simulink model "ds_simple_twozone"  (R2020a)
settings: Solver=ode1be  StartTime=0.0  StopTime=Inf  FixedStep=0.001  RelTol=1e-3
PostLoadFcn:
  | if any(exist('dsrtsu_mdlpostloadfcn', 'file') ~= 0), dsrtsu_mdlpostloadfcn('Execute', bdroot); end
InitFcn:
  | , if any(exist('rtifpga_mdlclblib', 'file') ~= 0), rtifpga_mdlclblib('Init', bdroot); end,
  | , if any(exist('dsmpb_private', 'file') ~= 0), dsmpb_private('dsmpb_mdlclblib', 'Init', bdroot); end,
libraries: neural x7, dsmpblib x7
(part 2 of 3)

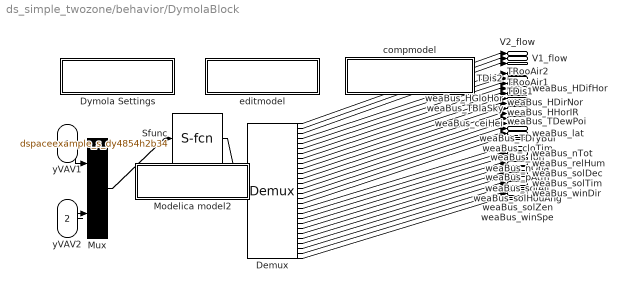
== system ds_simple_twozone/behavior/DymolaBlock ==
  yVAV1 : Inport
  yVAV2 : Inport  Port=2
  Demux : Demux  Outputs=[1;1;1;1;1;1;1;1;1;1;1;1;1;1;1;1;1;1;1;1;1;1;1;1;1;1;1;1]
  Dymola Settings : Subsystem  mask{ModelName=dSpaceExample.SimpleTwoZone, MoFileName=D:/github/dspace-modelica-example/dSpaceExample/SimpleTwoZone.mo, dSpace=, BusConnector=0, ResultFile=[], ResultFileOnline=[], ResultDt=[], Libs=:, bigobj=[], ImportFolder=[], guimode=[], ModelName2=[], forRuntime=[], MEXLoad=[], omitDescription=[], ResultName=dspaceexample_s_dy4854h2b34}
      mask prompts: ModelName "Name of Dymola model"; MoFileName "File Name (including .mo)"; ResultFile "Create Result"; ResultFileOnline "Load result"; ResultDt "Result min dt"; Libs "Used Libraries"; bigobj "Compiler flag /bigobj"; ImportFolder "Import folder"; guimode "GUI mode flag"; ModelName2 "Model name for import mode"; forRuntime "Runtime export"; MEXLoad "Compiled S-function"; omitDescription "Omit description strings"; ResultName "Name of result file"
      mask Display: disp('Dymola Settings');
  Modelica model2 : Subsystem
      mask Display: disp('Change parameters');
  Mux : Mux  Inputs=[1;1]
  Sfunc : S-Function  Tag=4854h2b34  FunctionName=dspaceexample_s_dy4854h2b34  Parameters=[VRoo;vav1_vav_sta_default_p;vav1_vav_sta_default_T;vav1_vav_sta_default_X;vav1_vav_riseTime;vav1_vav_y_start;vav1_vav_filter_gain;vav1_vav_filter_A_ripple;vav1_vav_filter_f_min;vav1_vav_filter_normalize10;vav1_vav_filter_x_start;vav1_vav_filter_u_nominal;vav1_vav_use_deltaM;vav1_vav_deltaM;vav1_vav_roundDuct;vav1_vav_ReC;vav1_vav_a;vav1_vav_b;vav1_vav_yL;vav1_vav_yU;vav1_vav_k1;vav1_vav_l;vav1_vav_l2;vav1_vav_deltax;vav1_vav_y_min;vav1_terHea_bal1_preDro_s26;vav1_terHea_bal1_preDro_s27;vav1_terHea_bal1_preDro_s28;vav1_terHea_bal2_preDro_s29;vav1_terHea_bal2_preDro_s30;vav1_terHea_delta;vav1_terHea_T_a1_nominal;vav1_terHea_T_a2_nominal;vav1_terHea_r_nominal;vav1_terHea_hA_n_w;vav1_terHea_hA_n_a;vav1_terHea_hA_T0_w;vav1_terHea_hA_T0_a;vav1_sinTer_X;vav1_sinTer_p;vav1_sinTer_T;vav1_souTer_X;vav1_souTer_m_flow;vav1_souTer_T;zer_k;zon1_S_;zon1_E_;zon1_W_;zon1_N_;zon1_matExtWal_absIR_a;zon1_matExtWal_absIR_b;zon1_matExtWal_absSol_a;zon1_matExtWal_absSol_b;zon1_matExtWal_roughness_54;zon1_matFlo_absIR_a;zon1_matFlo_absIR_b;zon1_matFlo_absSol_a;zon1_matFlo_absSol_b;zon1_matFlo_roughness_a;zon1_roof_absIR_a;zon1_roof_absIR_b;zon1_roof_absSol_a;zon1_roof_absSol_b;zon1_roof_roughness_a;zon1_window600_glass_1__x;zon1_window600_glass_1__k;zon1_window600_glass_1__t67;zon1_window600_glass_1__r68;zon1_window600_glass_1__r69;zon1_window600_glass_1__t70;zon1_window600_glass_1__a71;zon1_window600_glass_1__a72;zon1_window600_glass_2__x;zon1_window600_glass_2__k;zon1_window600_glass_2__t75;zon1_window600_glass_2__r76;zon1_window600_glass_2__r77;zon1_window600_glass_2__t78;zon1_window600_glass_2__a79;zon1_window600_glass_2__a80;zon1_window600_gas_1__x;zon1_window600_gas_1__a_k;zon1_window600_gas_1__b_k;zon1_window600_gas_1__a_m84;zon1_window600_gas_1__b_m85;zon1_window600_gas_1__a_c;zon1_window600_gas_1__b_c;zon1_window600_gas_1__MM;zon1_window600_gas_1__P0;zon1_window600_shade_tauS90;zon1_window600_shade_tauS91;zon1_window600_shade_rhoS92;zon1_window600_shade_rhoS93;zon1_window600_shade_absI94;zon1_window600_shade_absI95;zon1_window600_shade_tauI96;zon1_window600_shade_tauI97;zon1_window600_UFra;zon1_window600_absIRFra;zon1_window600_absSolFra;zon1_soi_A;zon1_soi_T_a_start;zon1_soi_T_b_start;zon1_roo_datConExt_1__bou104;zon1_roo_datConExt_1__A;zon1_roo_datConExt_2__bou106;zon1_roo_datConExt_2__A;zon1_roo_datConExt_3__bou108;zon1_roo_datConExt_3__A;zon1_roo_datConExt_4__bou110;zon1_roo_datConExt_4__A;zon1_roo_datConExtWin_1__112;zon1_roo_datConExtWin_1__113;zon1_roo_datConExtWin_1__114;zon1_roo_datConExtWin_1__115;zon1_roo_datConExtWin_1__116;zon1_roo_datConExtWin_1__117;zon1_roo_datConExtWin_1__118;zon1_roo_datConExtWin_1__119;zon1_roo_datConExtWin_1__120;zon1_roo_datConExtWin_1__121;zon1_roo_datConPar_1__azi;zon1_roo_datConPar_1__bou123;zon1_roo_datConPar_1__A;zon1_roo_datConBou_1__azi;zon1_roo_datConBou_1__bou126;zon1_roo_datConBou_1__A;zon1_roo_surBou_1__A;zon1_roo_surBou_1__absIR;zon1_roo_surBou_1__absSol;zon1_roo_surBou_1__bounda131;zon1_roo_dummyCon_absIR_a;zon1_roo_dummyCon_absIR_b;zon1_roo_dummyCon_absSol_134;zon1_roo_dummyCon_absSol_135;zon1_roo_dummyCon_roughne136;zon1_roo_dummyGlaSys_glas137;zon1_roo_dummyGlaSys_glas138;zon1_roo_dummyGlaSys_glas139;zon1_roo_dummyGlaSys_glas140;zon1_roo_dummyGlaSys_glas141;zon1_roo_dummyGlaSys_glas142;zon1_roo_dummyGlaSys_glas143;zon1_roo_dummyGlaSys_glas144;zon1_roo_dummyGlaSys_gas_145;zon1_roo_dummyGlaSys_gas_146;zon1_roo_dummyGlaSys_gas_147;zon1_roo_dummyGlaSys_gas_148;zon1_roo_dummyGlaSys_gas_149;zon1_roo_dummyGlaSys_gas_150;zon1_roo_dummyGlaSys_gas_151;zon1_roo_dummyGlaSys_gas_152;zon1_roo_dummyGlaSys_gas_153;zon1_roo_dummyGlaSys_shad154;zon1_roo_dummyGlaSys_shad155;zon1_roo_dummyGlaSys_shad156;zon1_roo_dummyGlaSys_shad157;zon1_roo_dummyGlaSys_shad158;zon1_roo_dummyGlaSys_shad159;zon1_roo_dummyGlaSys_shad160;zon1_roo_dummyGlaSys_shad161;zon1_roo_dummyGlaSys_UFra;zon1_roo_dummyGlaSys_absI163;zon1_roo_dummyGlaSys_absS164;zon1_roo_AFlo;zon1_roo_hRoo;zon1_roo_conExtWin_1__gla167;zon1_roo_conExtWin_1__win168;zon1_roo_conExtWin_1__win169;zon1_roo_conExtWin_1__win170;zon1_roo_conExtWin_1__win171;zon1_roo_hIntFixed;zon1_roo_hExtFixed;zon1_roo_bouConExt_HDifTi174;zon1_roo_bouConExt_HDifTi175;zon1_roo_bouConExt_HDifTi176;zon1_roo_bouConExt_HDifTi177;zon1_roo_bouConExt_HDifTi178;zon1_roo_bouConExt_HDifTi179;zon1_roo_bouConExt_HDifTi180;zon1_roo_bouConExt_HDifTi181;zon1_roo_bouConExt_HDifTi182;zon1_roo_bouConExt_HDifTi183;zon1_roo_bouConExt_HDifTi184;zon1_roo_bouConExt_HDifTi185;zon1_roo_bouConExtWin_con186;zon1_roo_bouConExtWin_con187;zon1_roo_bouConExtWin_HDi188;zon1_roo_bouConExtWin_HDi189;zon1_roo_bouConExtWin_HDi190;zon1_roo_bouConExtWin_con191;zon1_roo_air_datConExtWin192;zon1_roo_air_datConExtWin193;zon1_roo_air_dummyCon_abs194;zon1_roo_air_dummyCon_abs195;zon1_roo_air_dummyCon_abs196;zon1_roo_air_dummyCon_abs197;zon1_roo_air_dummyCon_rou198;zon1_roo_air_dummyGlaSys_199;zon1_roo_air_dummyGlaSys_200;zon1_roo_air_dummyGlaSys_201;zon1_roo_air_dummyGlaSys_202;zon1_roo_air_dummyGlaSys_203;zon1_roo_air_dummyGlaSys_204;zon1_roo_air_dummyGlaSys_205;zon1_roo_air_dummyGlaSys_206;zon1_roo_air_dummyGlaSys_207;zon1_roo_air_dummyGlaSys_208;zon1_roo_air_dummyGlaSys_209;zon1_roo_air_dummyGlaSys_210;zon1_roo_air_dummyGlaSys_211;zon1_roo_air_dummyGlaSys_212;zon1_roo_air_dummyGlaSys_213;zon1_roo_air_dummyGlaSys_214;zon1_roo_air_dummyGlaSys_215;zon1_roo_air_dummyGlaSys_216;zon1_roo_air_dummyGlaSys_217;zon1_roo_air_dummyGlaSys_218;zon1_roo_air_dummyGlaSys_219;zon1_roo_air_dummyGlaSys_220;zon1_roo_air_dummyGlaSys_221;zon1_roo_air_dummyGlaSys_222;zon1_roo_air_dummyGlaSys_223;zon1_roo_air_dummyGlaSys_224;zon1_roo_air_dummyGlaSys_225;zon1_roo_air_dummyGlaSys_226;zon1_roo_solRadExc_datCon227;zon1_roo_solRadExc_datCon228;zon1_roo_solRadExc_dummyC229;zon1_roo_solRadExc_dummyC230;zon1_roo_solRadExc_dummyC231;zon1_roo_solRadExc_dummyC232;zon1_roo_solRadExc_dummyC233;zon1_roo_solRadExc_dummyG234;zon1_roo_solRadExc_dummyG235;zon1_roo_solRadExc_dummyG236;zon1_roo_solRadExc_dummyG237;zon1_roo_solRadExc_dummyG238;zon1_roo_solRadExc_dummyG239;zon1_roo_solRadExc_dummyG240;zon1_roo_solRadExc_dummyG241;zon1_roo_solRadExc_dummyG242;zon1_roo_solRadExc_dummyG243;zon1_roo_solRadExc_dummyG244;zon1_roo_solRadExc_dummyG245;zon1_roo_solRadExc_dummyG246;zon1_roo_solRadExc_dummyG247;zon1_roo_solRadExc_dummyG248;zon1_roo_solRadExc_dummyG249;zon1_roo_solRadExc_dummyG250;zon1_roo_solRadExc_dummyG251;zon1_roo_solRadExc_dummyG252;zon1_roo_solRadExc_dummyG253;zon1_roo_solRadExc_dummyG254;zon1_roo_solRadExc_dummyG255;zon1_roo_solRadExc_dummyG256;zon1_roo_solRadExc_dummyG257;zon1_roo_solRadExc_dummyG258;zon1_roo_solRadExc_dummyG259;zon1_roo_solRadExc_dummyG260;zon1_roo_solRadExc_dummyG261;zon1_roo_irRadGai_datConE262;zon1_roo_irRadGai_datConE263;zon1_roo_irRadGai_dummyCo264;zon1_roo_irRadGai_dummyCo265;zon1_roo_irRadGai_dummyCo266;zon1_roo_irRadGai_dummyCo267;zon1_roo_irRadGai_dummyCo268;zon1_roo_irRadGai_dummyGl269;zon1_roo_irRadGai_dummyGl270;zon1_roo_irRadGai_dummyGl271;zon1_roo_irRadGai_dummyGl272;zon1_roo_irRadGai_dummyGl273;zon1_roo_irRadGai_dummyGl274;zon1_roo_irRadGai_dummyGl275;zon1_roo_irRadGai_dummyGl276;zon1_roo_irRadGai_dummyGl277;zon1_roo_irRadGai_dummyGl278;zon1_roo_irRadGai_dummyGl279;zon1_roo_irRadGai_dummyGl280;zon1_roo_irRadGai_dummyGl281;zon1_roo_irRadGai_dummyGl282;zon1_roo_irRadGai_dummyGl283;zon1_roo_irRadGai_dummyGl284;zon1_roo_irRadGai_dummyGl285;zon1_roo_irRadGai_dummyGl286;zon1_roo_irRadGai_dummyGl287;zon1_roo_irRadGai_dummyGl288;zon1_roo_irRadGai_dummyGl289;zon1_roo_irRadGai_dummyGl290;zon1_roo_irRadGai_dummyGl291;zon1_roo_irRadGai_dummyGl292;zon1_roo_irRadGai_dummyGl293;zon1_roo_irRadGai_dummyGl294;zon1_roo_irRadGai_dummyGl295;zon1_roo_irRadGai_dummyGl296;zon1_roo_irRadExc_datConE297;zon1_roo_irRadExc_datConE298;zon1_roo_irRadExc_dummyCo299;zon1_roo_irRadExc_dummyCo300;zon1_roo_irRadExc_dummyCo301;zon1_roo_irRadExc_dummyCo302;zon1_roo_irRadExc_dummyCo303;zon1_roo_irRadExc_dummyGl304;zon1_roo_irRadExc_dummyGl305;zon1_roo_irRadExc_dummyGl306;zon1_roo_irRadExc_dummyGl307;zon1_roo_irRadExc_dummyGl308;zon1_roo_irRadExc_dummyGl309;zon1_roo_irRadExc_dummyGl310;zon1_roo_irRadExc_dummyGl311;zon1_roo_irRadExc_dummyGl312;zon1_roo_irRadExc_dummyGl313;zon1_roo_irRadExc_dummyGl314;zon1_roo_irRadExc_dummyGl315;zon1_roo_irRadExc_dummyGl316;zon1_roo_irRadExc_dummyGl317;zon1_roo_irRadExc_dummyGl318;zon1_roo_irRadExc_dummyGl319;zon1_roo_irRadExc_dummyGl320;zon1_roo_irRadExc_dummyGl321;zon1_roo_irRadExc_dummyGl322;zon1_roo_irRadExc_dummyGl323;zon1_roo_irRadExc_dummyGl324;zon1_roo_irRadExc_dummyGl325;zon1_roo_irRadExc_dummyGl326;zon1_roo_irRadExc_dummyGl327;zon1_roo_irRadExc_dummyGl328;zon1_roo_irRadExc_dummyGl329;zon1_roo_irRadExc_dummyGl330;zon1_roo_irRadExc_dummyGl331;zon1_roo_irRadExc_T0;zon1_roo_radTem_datConExt333;zon1_roo_radTem_datConExt334;zon1_roo_radTem_dummyCon_335;zon1_roo_radTem_dummyCon_336;zon1_roo_radTem_dummyCon_337;zon1_roo_radTem_dummyCon_338;zon1_roo_radTem_dummyCon_339;zon1_roo_radTem_dummyGlaS340;zon1_roo_radTem_dummyGlaS341;zon1_roo_radTem_dummyGlaS342;zon1_roo_radTem_dummyGlaS343;zon1_roo_radTem_dummyGlaS344;zon1_roo_radTem_dummyGlaS345;zon1_roo_radTem_dummyGlaS346;zon1_roo_radTem_dummyGlaS347;zon1_roo_radTem_dummyGlaS348;zon1_roo_radTem_dummyGlaS349;zon1_roo_radTem_dummyGlaS350;zon1_roo_radTem_dummyGlaS351;zon1_roo_radTem_dummyGlaS352;zon1_roo_radTem_dummyGlaS353;zon1_roo_radTem_dummyGlaS354;zon1_roo_radTem_dummyGlaS355;zon1_roo_radTem_dummyGlaS356;zon1_roo_radTem_dummyGlaS357;zon1_roo_radTem_dummyGlaS358;zon1_roo_radTem_dummyGlaS359;zon1_roo_radTem_dummyGlaS360;zon1_roo_radTem_dummyGlaS361;zon1_roo_radTem_dummyGlaS362;zon1_roo_radTem_dummyGlaS363;zon1_roo_radTem_dummyGlaS364;zon1_roo_radTem_dummyGlaS365;zon1_roo_radTem_dummyGlaS366;zon1_roo_radTem_dummyGlaS367;zon1_roo_add_k1;zon1_roo_add_k2;zon1_roo_sumJFroWin_1__k;zon1_roo_p_start;zon1_roo_T_start;zon1_roo_X_start;zon1_qConGai_flow_k;zon1_qRadGai_flow_k;zon1_qLatGai_flow_k;zon1_TSoi_1__T;zon1_sinInf_m_flow;zon1_sinInf_x_pTphi_p;zon1_InfiltrationRate_k;zon1_souInf_m_flow;zon1_souInf_x_pTphi_p;zon1_intLoad_table;zon1_intLoad_verboseRead;zon1_intLoad_columns;zon1_intLoad_offset;zon1_intLoad_startTime;zon1_intLoad_timeEvents;weaDat_pAtm;weaDat_TDryBul;weaDat_TDewPoi;weaDat_TBlaSky;weaDat_relHum;weaDat_winSpe;weaDat_winDir;weaDat_HInfHor;weaDat_ceiHei;weaDat_totSkyCov;weaDat_opaSkyCov;weaDat_datRea_verboseRead;weaDat_cheTemDryBul_TMin;weaDat_cheTemDryBul_TMax;weaDat_cheTemDewPoi_TMin;weaDat_cheTemDewPoi_TMax;weaDat_add30Min_k1;weaDat_add30Min_k2;weaDat_datRea30Min_verbos407;weaDat_cheTemBlaSky_TMin;weaDat_cheTemBlaSky_TMax;rooSin_p;rooSin_T;rooSin_X;zon2_S_;zon2_E_;zon2_W_;zon2_N_;zon2_matExtWal_absIR_a;zon2_matExtWal_absIR_b;zon2_matExtWal_absSol_a;zon2_matExtWal_absSol_b;zon2_matExtWal_roughness_421;zon2_matFlo_absIR_a;zon2_matFlo_absIR_b;zon2_matFlo_absSol_a;zon2_matFlo_absSol_b;zon2_matFlo_roughness_a;zon2_roof_absIR_a;zon2_roof_absIR_b;zon2_roof_absSol_a;zon2_roof_absSol_b;zon2_roof_roughness_a;zon2_window600_glass_1__x;zon2_window600_glass_1__k;zon2_window600_glass_1__t434;zon2_window600_glass_1__r435;zon2_window600_glass_1__r436;zon2_window600_glass_1__t437;zon2_window600_glass_1__a438;zon2_window600_glass_1__a439;zon2_window600_glass_2__x;zon2_window600_glass_2__k;zon2_window600_glass_2__t442;zon2_window600_glass_2__r443;zon2_window600_glass_2__r444;zon2_window600_glass_2__t445;zon2_window600_glass_2__a446;zon2_window600_glass_2__a447;zon2_window600_gas_1__x;zon2_window600_gas_1__a_k;zon2_window600_gas_1__b_k;zon2_window600_gas_1__a_m451;zon2_window600_gas_1__b_m452;zon2_window600_gas_1__a_c;zon2_window600_gas_1__b_c;zon2_window600_gas_1__MM;zon2_window600_gas_1__P0;zon2_window600_shade_tauS457;zon2_window600_shade_tauS458;zon2_window600_shade_rhoS459;zon2_window600_shade_rhoS460;zon2_window600_shade_absI461;zon2_window600_shade_absI462;zon2_window600_shade_tauI463;zon2_window600_shade_tauI464;zon2_window600_UFra;zon2_window600_absIRFra;zon2_window600_absSolFra;zon2_soi_A;zon2_soi_T_a_start;zon2_soi_T_b_start;zon2_roo_datConExt_1__bou471;zon2_roo_datConExt_1__A;zon2_roo_datConExt_2__bou473;zon2_roo_datConExt_2__A;zon2_roo_datConExt_3__bou475;zon2_roo_datConExt_3__A;zon2_roo_datConExt_4__bou477;zon2_roo_datConExt_4__A;zon2_roo_datConExtWin_1__479;zon2_roo_datConExtWin_1__480;zon2_roo_datConExtWin_1__481;zon2_roo_datConExtWin_1__482;zon2_roo_datConExtWin_1__483;zon2_roo_datConExtWin_1__484;zon2_roo_datConExtWin_1__485;zon2_roo_datConExtWin_1__486;zon2_roo_datConExtWin_1__487;zon2_roo_datConExtWin_1__488;zon2_roo_datConPar_1__azi;zon2_roo_datConPar_1__bou490;zon2_roo_datConPar_1__A;zon2_roo_datConBou_1__azi;zon2_roo_datConBou_1__bou493;zon2_roo_datConBou_1__A;zon2_roo_surBou_1__A;zon2_roo_surBou_1__absIR;zon2_roo_surBou_1__absSol;zon2_roo_surBou_1__bounda498;zon2_roo_dummyCon_absIR_a;zon2_roo_dummyCon_absIR_b;zon2_roo_dummyCon_absSol_501;zon2_roo_dummyCon_absSol_502;zon2_roo_dummyCon_roughne503;zon2_roo_dummyGlaSys_glas504;zon2_roo_dummyGlaSys_glas505;zon2_roo_dummyGlaSys_glas506;zon2_roo_dummyGlaSys_glas507;zon2_roo_dummyGlaSys_glas508;zon2_roo_dummyGlaSys_glas509;zon2_roo_dummyGlaSys_glas510;zon2_roo_dummyGlaSys_glas511;zon2_roo_dummyGlaSys_gas_512;zon2_roo_dummyGlaSys_gas_513;zon2_roo_dummyGlaSys_gas_514;zon2_roo_dummyGlaSys_gas_515;zon2_roo_dummyGlaSys_gas_516;zon2_roo_dummyGlaSys_gas_517;zon2_roo_dummyGlaSys_gas_518;zon2_roo_dummyGlaSys_gas_519;zon2_roo_dummyGlaSys_gas_520;zon2_roo_dummyGlaSys_shad521;zon2_roo_dummyGlaSys_shad522;zon2_roo_dummyGlaSys_shad523;zon2_roo_dummyGlaSys_shad524;zon2_roo_dummyGlaSys_shad525;zon2_roo_dummyGlaSys_shad526;zon2_roo_dummyGlaSys_shad527;zon2_roo_dummyGlaSys_shad528;zon2_roo_dummyGlaSys_UFra;zon2_roo_dummyGlaSys_absI530;zon2_roo_dummyGlaSys_absS531;zon2_roo_AFlo;zon2_roo_hRoo;zon2_roo_conExtWin_1__gla534;zon2_roo_conExtWin_1__win535;zon2_roo_conExtWin_1__win536;zon2_roo_conExtWin_1__win537;zon2_roo_conExtWin_1__win538;zon2_roo_hIntFixed;zon2_roo_hExtFixed;zon2_roo_bouConExt_HDifTi541;zon2_roo_bouConExt_HDifTi542;zon2_roo_bouConExt_HDifTi543;zon2_roo_bouConExt_HDifTi544;zon2_roo_bouConExt_HDifTi545;zon2_roo_bouConExt_HDifTi546;zon2_roo_bouConExt_HDifTi547;zon2_roo_bouConExt_HDifTi548;zon2_roo_bouConExt_HDifTi549;zon2_roo_bouConExt_HDifTi550;zon2_roo_bouConExt_HDifTi551;zon2_roo_bouConExt_HDifTi552;zon2_roo_bouConExtWin_con553;zon2_roo_bouConExtWin_con554;zon2_roo_bouConExtWin_HDi555;zon2_roo_bouConExtWin_HDi556;zon2_roo_bouConExtWin_HDi557;zon2_roo_bouConExtWin_con558;zon2_roo_air_datConExtWin559;zon2_roo_air_datConExtWin560;zon2_roo_air_dummyCon_abs561;zon2_roo_air_dummyCon_abs562;zon2_roo_air_dummyCon_abs563;zon2_roo_air_dummyCon_abs564;zon2_roo_air_dummyCon_rou565;zon2_roo_air_dummyGlaSys_566;zon2_roo_air_dummyGlaSys_567;zon2_roo_air_dummyGlaSys_568;zon2_roo_air_dummyGlaSys_569;zon2_roo_air_dummyGlaSys_570;zon2_roo_air_dummyGlaSys_571;zon2_roo_air_dummyGlaSys_572;zon2_roo_air_dummyGlaSys_573;zon2_roo_air_dummyGlaSys_574;zon2_roo_air_dummyGlaSys_575;zon2_roo_air_dummyGlaSys_576;zon2_roo_air_dummyGlaSys_577;zon2_roo_air_dummyGlaSys_578;zon2_roo_air_dummyGlaSys_579;zon2_roo_air_dummyGlaSys_580;zon2_roo_air_dummyGlaSys_581;zon2_roo_air_dummyGlaSys_582;zon2_roo_air_dummyGlaSys_583;zon2_roo_air_dummyGlaSys_584;zon2_roo_air_dummyGlaSys_585;zon2_roo_air_dummyGlaSys_586;zon2_roo_air_dummyGlaSys_587;zon2_roo_air_dummyGlaSys_588;zon2_roo_air_dummyGlaSys_589;zon2_roo_air_dummyGlaSys_590;zon2_roo_air_dummyGlaSys_591;zon2_roo_air_dummyGlaSys_592;zon2_roo_air_dummyGlaSys_593;zon2_roo_solRadExc_datCon594;zon2_roo_solRadExc_datCon595;zon2_roo_solRadExc_dummyC596;zon2_roo_solRadExc_dummyC597;zon2_roo_solRadExc_dummyC598;zon2_roo_solRadExc_dummyC599;zon2_roo_solRadExc_dummyC600;zon2_roo_solRadExc_dummyG601;zon2_roo_solRadExc_dummyG602;zon2_roo_solRadExc_dummyG603;zon2_roo_solRadExc_dummyG604;zon2_roo_solRadExc_dummyG605;zon2_roo_solRadExc_dummyG606;zon2_roo_solRadExc_dummyG607;zon2_roo_solRadExc_dummyG608;zon2_roo_solRadExc_dummyG609;zon2_roo_solRadExc_dummyG610;zon2_roo_solRadExc_dummyG611;zon2_roo_solRadExc_dummyG612;zon2_roo_solRadExc_dummyG613;zon2_roo_solRadExc_dummyG614;zon2_roo_solRadExc_dummyG615;zon2_roo_solRadExc_dummyG616;zon2_roo_solRadExc_dummyG617;zon2_roo_solRadExc_dummyG618;zon2_roo_solRadExc_dummyG619;zon2_roo_solRadExc_dummyG620;zon2_roo_solRadExc_dummyG621;zon2_roo_solRadExc_dummyG622;zon2_roo_solRadExc_dummyG623;zon2_roo_solRadExc_dummyG624;zon2_roo_solRadExc_dummyG625;zon2_roo_solRadExc_dummyG626;zon2_roo_solRadExc_dummyG627;zon2_roo_solRadExc_dummyG628;zon2_roo_irRadGai_datConE629;zon2_roo_irRadGai_datConE630;zon2_roo_irRadGai_dummyCo631;zon2_roo_irRadGai_dummyCo632;zon2_roo_irRadGai_dummyCo633;zon2_roo_irRadGai_dummyCo634;zon2_roo_irRadGai_dummyCo635;zon2_roo_irRadGai_dummyGl636;zon2_roo_irRadGai_dummyGl637;zon2_roo_irRadGai_dummyGl638;zon2_roo_irRadGai_dummyGl639;zon2_roo_irRadGai_dummyGl640;zon2_roo_irRadGai_dummyGl641;zon2_roo_irRadGai_dummyGl642;zon2_roo_irRadGai_dummyGl643;zon2_roo_irRadGai_dummyGl644;zon2_roo_irRadGai_dummyGl645;zon2_roo_irRadGai_dummyGl646;zon2_roo_irRadGai_dummyGl647;zon2_roo_irRadGai_dummyGl648;zon2_roo_irRadGai_dummyGl649;zon2_roo_irRadGai_dummyGl650;zon2_roo_irRadGai_dummyGl651;zon2_roo_irRadGai_dummyGl652;zon2_roo_irRadGai_dummyGl653;zon2_roo_irRadGai_dummyGl654;zon2_roo_irRadGai_dummyGl655;zon2_roo_irRadGai_dummyGl656;zon2_roo_irRadGai_dummyGl657;zon2_roo_irRadGai_dummyGl658;zon2_roo_irRadGai_dummyGl659;zon2_roo_irRadGai_dummyGl660;zon2_roo_irRadGai_dummyGl661;zon2_roo_irRadGai_dummyGl662;zon2_roo_irRadGai_dummyGl663;zon2_roo_irRadExc_datConE664;zon2_roo_irRadExc_datConE665;zon2_roo_irRadExc_dummyCo666;zon2_roo_irRadExc_dummyCo667;zon2_roo_irRadExc_dummyCo668;zon2_roo_irRadExc_dummyCo669;zon2_roo_irRadExc_dummyCo670;zon2_roo_irRadExc_dummyGl671;zon2_roo_irRadExc_dummyGl672;zon2_roo_irRadExc_dummyGl673;zon2_roo_irRadExc_dummyGl674;zon2_roo_irRadExc_dummyGl675;zon2_roo_irRadExc_dummyGl676;zon2_roo_irRadExc_dummyGl677;zon2_roo_irRadExc_dummyGl678;zon2_roo_irRadExc_dummyGl679;zon2_roo_irRadExc_dummyGl680;zon2_roo_irRadExc_dummyGl681;zon2_roo_irRadExc_dummyGl682;zon2_roo_irRadExc_dummyGl683;zon2_roo_irRadExc_dummyGl684;zon2_roo_irRadExc_dummyGl685;zon2_roo_irRadExc_dummyGl686;zon2_roo_irRadExc_dummyGl687;zon2_roo_irRadExc_dummyGl688;zon2_roo_irRadExc_dummyGl689;zon2_roo_irRadExc_dummyGl690;zon2_roo_irRadExc_dummyGl691;zon2_roo_irRadExc_dummyGl692;zon2_roo_irRadExc_dummyGl693;zon2_roo_irRadExc_dummyGl694;zon2_roo_irRadExc_dummyGl695;zon2_roo_irRadExc_dummyGl696;zon2_roo_irRadExc_dummyGl697;zon2_roo_irRadExc_dummyGl698;zon2_roo_irRadExc_T0;zon2_roo_radTem_datConExt700;zon2_roo_radTem_datConExt701;zon2_roo_radTem_dummyCon_702;zon2_roo_radTem_dummyCon_703;zon2_roo_radTem_dummyCon_704;zon2_roo_radTem_dummyCon_705;zon2_roo_radTem_dummyCon_706;zon2_roo_radTem_dummyGlaS707;zon2_roo_radTem_dummyGlaS708;zon2_roo_radTem_dummyGlaS709;zon2_roo_radTem_dummyGlaS710;zon2_roo_radTem_dummyGlaS711;zon2_roo_radTem_dummyGlaS712;zon2_roo_radTem_dummyGlaS713;zon2_roo_radTem_dummyGlaS714;zon2_roo_radTem_dummyGlaS715;zon2_roo_radTem_dummyGlaS716;zon2_roo_radTem_dummyGlaS717;zon2_roo_radTem_dummyGlaS718;zon2_roo_radTem_dummyGlaS719;zon2_roo_radTem_dummyGlaS720;zon2_roo_radTem_dummyGlaS721;zon2_roo_radTem_dummyGlaS722;zon2_roo_radTem_dummyGlaS723;zon2_roo_radTem_dummyGlaS724;zon2_roo_radTem_dummyGlaS725;zon2_roo_radTem_dummyGlaS726;zon2_roo_radTem_dummyGlaS727;zon2_roo_radTem_dummyGlaS728;zon2_roo_radTem_dummyGlaS729;zon2_roo_radTem_dummyGlaS730;zon2_roo_radTem_dummyGlaS731;zon2_roo_radTem_dummyGlaS732;zon2_roo_radTem_dummyGlaS733;zon2_roo_radTem_dummyGlaS734;zon2_roo_add_k1;zon2_roo_add_k2;zon2_roo_sumJFroWin_1__k;zon2_roo_p_start;zon2_roo_T_start;zon2_roo_X_start;zon2_qConGai_flow_k;zon2_qRadGai_flow_k;zon2_qLatGai_flow_k;zon2_TSoi_1__T;zon2_sinInf_m_flow;zon2_sinInf_x_pTphi_p;zon2_InfiltrationRate_k;zon2_souInf_m_flow;zon2_souInf_x_pTphi_p;zon2_intLoad_table;zon2_intLoad_verboseRead;zon2_intLoad_columns;zon2_intLoad_offset;zon2_intLoad_startTime;zon2_intLoad_timeEvents;vav2_vav_sta_default_p;vav2_vav_sta_default_T;vav2_vav_sta_default_X;vav2_vav_riseTime;vav2_vav_y_start;vav2_vav_filter_gain;vav2_vav_filter_A_ripple;vav2_vav_filter_f_min;vav2_vav_filter_normalize764;vav2_vav_filter_x_start;vav2_vav_filter_u_nominal;vav2_vav_use_deltaM;vav2_vav_deltaM;vav2_vav_roundDuct;vav2_vav_ReC;vav2_vav_a;vav2_vav_b;vav2_vav_yL;vav2_vav_yU;vav2_vav_k1;vav2_vav_l;vav2_vav_l2;vav2_vav_deltax;vav2_vav_y_min;vav2_terHea_bal1_preDro_s780;vav2_terHea_bal1_preDro_s781;vav2_terHea_bal1_preDro_s782;vav2_terHea_bal2_preDro_s783;vav2_terHea_bal2_preDro_s784;vav2_terHea_delta;vav2_terHea_T_a1_nominal;vav2_terHea_T_a2_nominal;vav2_terHea_r_nominal;vav2_terHea_hA_n_w;vav2_terHea_hA_n_a;vav2_terHea_hA_T0_w;vav2_terHea_hA_T0_a;vav2_sinTer_X;vav2_sinTer_p;vav2_sinTer_T;vav2_souTer_X;vav2_souTer_m_flow;vav2_souTer_T;coiSou_X;coiSou_T;byp_sta_default_p;byp_sta_default_T;byp_sta_default_X;VSup2_T_start;VSup2_p_start;VSup2_X_start;VSup1_T_start;VSup1_p_start;VSup1_X_start;TDisVAV1_T_start;TDisVAV1_TAmb;TDisVAV1_tauHeaTra;TDisVAV2_T_start;TDisVAV2_TAmb;TDisVAV2_tauHeaTra;zon1_roo_conExtWin_1__win816;zon1_roo_conExtWin_1__win817;zon1_roo_conExtWin_1__win818;zon2_roo_conExtWin_1__win819;zon2_roo_conExtWin_1__win820;zon2_roo_conExtWin_1__win821],[]  PortCounts=[1;1]  SFunctionDeploymentMode=off  EnableBusSupport=off  mask{VRoo=129.6, vav1_vav_sta_default_p=101325, vav1_vav_sta_default_T=293.15, vav1_vav_sta_default_X=[0.01; 0.99], vav1_vav_riseTime=120, vav1_vav_y_start=1, vav1_vav_filter_gain=1, vav1_vav_filter_A_ripple=0.5, vav1_vav_filter_f_min=0, vav1_vav_filter_normalize10=1, vav1_vav_filter_x_start=[0; 0], vav1_vav_filter_u_nominal=1, vav1_vav_use_deltaM=1, vav1_vav_deltaM=0.3, vav1_vav_roundDuct=0, vav1_vav_ReC=4000, vav1_vav_a=-1.51, vav1_vav_b=9.45, vav1_vav_yL=0.166666666666667, vav1_vav_yU=0.611111111111111, vav1_vav_k1=0.45, vav1_vav_l=0.0001, vav1_vav_l2=0.01, vav1_vav_deltax=0.02, vav1_vav_y_min=0.02, vav1_terHea_bal1_preDro_s26=101325, vav1_terHea_bal1_preDro_s27=293.15, vav1_terHea_bal1_preDro_s28=[0.01; 0.99], vav1_terHea_bal2_preDro_s29=300000, vav1_terHea_bal2_preDro_s30=293.15, vav1_terHea_delta=0.001, vav1_terHea_T_a1_nominal=289.85, vav1_terHea_T_a2_nominal=355.35, vav1_terHea_r_nominal=0.666666666666667, vav1_terHea_hA_n_w=0.85, vav1_terHea_hA_n_a=0.8, vav1_terHea_hA_T0_w=293.15, vav1_terHea_hA_T0_a=293.15, vav1_sinTer_X=1, vav1_sinTer_p=300000, vav1_sinTer_T=293.15, vav1_souTer_X=1, vav1_souTer_m_flow=0, vav1_souTer_T=323.15, zer_k=0, zon1_S_=0, zon1_E_=-1.5707963267949, zon1_W_=1.5707963267949, zon1_N_=3.14159265358979, zon1_matExtWal_absIR_a=0.9, zon1_matExtWal_absIR_b=0.9, zon1_matExtWal_absSol_a=0.6, zon1_matExtWal_absSol_b=0.6, zon1_matExtWal_roughness_54=3, zon1_matFlo_absIR_a=0.9, zon1_matFlo_absIR_b=0.9, zon1_matFlo_absSol_a=0.6, zon1_matFlo_absSol_b=0.6, zon1_matFlo_roughness_a=3, zon1_roof_absIR_a=0.9, zon1_roof_absIR_b=0.9, zon1_roof_absSol_a=0.6, zon1_roof_absSol_b=0.6, zon1_roof_roughness_a=3, zon1_window600_glass_1__x=0.003175, zon1_window600_glass_1__k=1.06, zon1_window600_glass_1__t67=0.86156, zon1_window600_glass_1__r68=0.0434, zon1_window600_glass_1__r69=0.0434, zon1_window600_glass_1__t70=0, zon1_window600_glass_1__a71=0.9, zon1_window600_glass_1__a72=0.9, zon1_window600_glass_2__x=0.003175, zon1_window600_glass_2__k=1.06, zon1_window600_glass_2__t75=0.86156, zon1_window600_glass_2__r76=0.0434, zon1_window600_glass_2__r77=0.0434, zon1_window600_glass_2__t78=0, zon1_window600_glass_2__a79=0.9, zon1_window600_glass_2__a80=0.9, zon1_window600_gas_1__x=0.013, zon1_window600_gas_1__a_k=0.002873, zon1_window600_gas_1__b_k=7.76e-05, zon1_window600_gas_1__a_m84=3.723e-06, zon1_window600_gas_1__b_m85=4.94e-08, zon1_window600_gas_1__a_c=1002.737, zon1_window600_gas_1__b_c=0.012324, zon1_window600_gas_1__MM=0.02897, zon1_window600_gas_1__P0=101325, zon1_window600_shade_tauS90=0.1, zon1_window600_shade_tauS91=0.1, zon1_window600_shade_rhoS92=0.8, zon1_window600_shade_rhoS93=0.8, zon1_window600_shade_absI94=0.84, zon1_window600_shade_absI95=0.84, zon1_window600_shade_tauI96=0, zon1_window600_shade_tauI97=0, zon1_window600_UFra=3, zon1_window600_absIRFra=0.8, zon1_window600_absSolFra=0.5, zon1_soi_A=48, zon1_soi_T_a_start=283.15, zon1_soi_T_b_start=283.75, zon1_roo_datConExt_1__bou104=1, zon1_roo_datConExt_1__A=48, zon1_roo_datConExt_2__bou106=1, zon1_roo_datConExt_2__A=16.2, zon1_roo_datConExt_3__bou108=1, zon1_roo_datConExt_3__A=16.2, zon1_roo_datConExt_4__bou110=1, zon1_roo_datConExt_4__A=21.6, zon1_roo_datConExtWin_1__112=1, zon1_roo_datConExtWin_1__113=21.6, zon1_roo_datConExtWin_1__114=2, zon1_roo_datConExtWin_1__115=6, zon1_roo_datConExtWin_1__116=0.001, zon1_roo_datConExtWin_1__117=0, zon1_roo_datConExtWin_1__118=0, zon1_roo_datConExtWin_1__119=0, zon1_roo_datConExtWin_1__120=0, zon1_roo_datConExtWin_1__121=0, zon1_roo_datConPar_1__azi=0, zon1_roo_datConPar_1__bou123=1, zon1_roo_datConPar_1__A=0, zon1_roo_datConBou_1__azi=0, zon1_roo_datConBou_1__bou126=1, zon1_roo_datConBou_1__A=48, zon1_roo_surBou_1__A=0, zon1_roo_surBou_1__absIR=0.84, zon1_roo_surBou_1__absSol=0.84, zon1_roo_surBou_1__bounda131=1, zon1_roo_dummyCon_absIR_a=0.9, zon1_roo_dummyCon_absIR_b=0.9, zon1_roo_dummyCon_absSol_134=0.5, zon1_roo_dummyCon_absSol_135=0.5, zon1_roo_dummyCon_roughne136=3, zon1_roo_dummyGlaSys_glas137=0.003, zon1_roo_dummyGlaSys_glas138=1, zon1_roo_dummyGlaSys_glas139=0.834, zon1_roo_dummyGlaSys_glas140=0.075, zon1_roo_dummyGlaSys_glas141=0.075, zon1_roo_dummyGlaSys_glas142=0, zon1_roo_dummyGlaSys_glas143=0.84, zon1_roo_dummyGlaSys_glas144=0.84, zon1_roo_dummyGlaSys_gas_145=-1, zon1_roo_dummyGlaSys_gas_146=0.002873, zon1_roo_dummyGlaSys_gas_147=7.76e-05, zon1_roo_dummyGlaSys_gas_148=3.723e-06, zon1_roo_dummyGlaSys_gas_149=4.94e-08, zon1_roo_dummyGlaSys_gas_150=1002.737, zon1_roo_dummyGlaSys_gas_151=0.012324, zon1_roo_dummyGlaSys_gas_152=0.02897, zon1_roo_dummyGlaSys_gas_153=101325, zon1_roo_dummyGlaSys_shad154=0.1, zon1_roo_dummyGlaSys_shad155=0.1, zon1_roo_dummyGlaSys_shad156=0.8, zon1_roo_dummyGlaSys_shad157=0.8, zon1_roo_dummyGlaSys_shad158=0.84, zon1_roo_dummyGlaSys_shad159=0.84, zon1_roo_dummyGlaSys_shad160=0, zon1_roo_dummyGlaSys_shad161=0, zon1_roo_dummyGlaSys_UFra=3, zon1_roo_dummyGlaSys_absI163=0.8, zon1_roo_dummyGlaSys_absS164=0.5, zon1_roo_AFlo=48, zon1_roo_hRoo=2.7, zon1_roo_conExtWin_1__gla167=0, zon1_roo_conExtWin_1__win168=1, zon1_roo_conExtWin_1__win169=3, zon1_roo_conExtWin_1__win170=331.4, zon1_roo_conExtWin_1__win171=1, zon1_roo_hIntFixed=3, zon1_roo_hExtFixed=10, zon1_roo_bouConExt_HDifTi174=0.2, zon1_roo_bouConExt_HDifTi175=1, zon1_roo_bouConExt_HDifTi176=1, zon1_roo_bouConExt_HDifTi177=0.2, zon1_roo_bouConExt_HDifTi178=1, zon1_roo_bouConExt_HDifTi179=1, zon1_roo_bouConExt_HDifTi180=0.2, zon1_roo_bouConExt_HDifTi181=1, zon1_roo_bouConExt_HDifTi182=1, zon1_roo_bouConExt_HDifTi183=0.2, zon1_roo_bouConExt_HDifTi184=1, zon1_roo_bouConExt_HDifTi185=1, zon1_roo_bouConExtWin_con186=0, zon1_roo_bouConExtWin_con187=0, zon1_roo_bouConExtWin_HDi188=0.2, zon1_roo_bouConExtWin_HDi189=1, zon1_roo_bouConExtWin_HDi190=1, zon1_roo_bouConExtWin_con191=293.15, zon1_roo_air_datConExtWin192=0, zon1_roo_air_datConExtWin193=0, zon1_roo_air_dummyCon_abs194=0.9, zon1_roo_air_dummyCon_abs195=0.9, zon1_roo_air_dummyCon_abs196=0.5, zon1_roo_air_dummyCon_abs197=0.5, zon1_roo_air_dummyCon_rou198=3, zon1_roo_air_dummyGlaSys_199=0.003, zon1_roo_air_dummyGlaSys_200=1, zon1_roo_air_dummyGlaSys_201=0.834, zon1_roo_air_dummyGlaSys_202=0.075, zon1_roo_air_dummyGlaSys_203=0.075, zon1_roo_air_dummyGlaSys_204=0, zon1_roo_air_dummyGlaSys_205=0.84, zon1_roo_air_dummyGlaSys_206=0.84, zon1_roo_air_dummyGlaSys_207=-1, zon1_roo_air_dummyGlaSys_208=0.002873, zon1_roo_air_dummyGlaSys_209=7.76e-05, zon1_roo_air_dummyGlaSys_210=3.723e-06, zon1_roo_air_dummyGlaSys_211=4.94e-08, zon1_roo_air_dummyGlaSys_212=1002.737, zon1_roo_air_dummyGlaSys_213=0.012324, zon1_roo_air_dummyGlaSys_214=0.02897, zon1_roo_air_dummyGlaSys_215=101325, zon1_roo_air_dummyGlaSys_216=0.1, zon1_roo_air_dummyGlaSys_217=0.1, zon1_roo_air_dummyGlaSys_218=0.8, zon1_roo_air_dummyGlaSys_219=0.8, zon1_roo_air_dummyGlaSys_220=0.84, zon1_roo_air_dummyGlaSys_221=0.84, zon1_roo_air_dummyGlaSys_222=0, zon1_roo_air_dummyGlaSys_223=0, zon1_roo_air_dummyGlaSys_224=3, zon1_roo_air_dummyGlaSys_225=0.8, zon1_roo_air_dummyGlaSys_226=0.5, zon1_roo_solRadExc_datCon227=0, zon1_roo_solRadExc_datCon228=0, zon1_roo_solRadExc_dummyC229=0.9, zon1_roo_solRadExc_dummyC230=0.9, zon1_roo_solRadExc_dummyC231=0.5, zon1_roo_solRadExc_dummyC232=0.5, zon1_roo_solRadExc_dummyC233=3, zon1_roo_solRadExc_dummyG234=0.003, zon1_roo_solRadExc_dummyG235=1, zon1_roo_solRadExc_dummyG236=0.834, zon1_roo_solRadExc_dummyG237=0.075, zon1_roo_solRadExc_dummyG238=0.075, zon1_roo_solRadExc_dummyG239=0, zon1_roo_solRadExc_dummyG240=0.84, zon1_roo_solRadExc_dummyG241=0.84, zon1_roo_solRadExc_dummyG242=-1, zon1_roo_solRadExc_dummyG243=0.002873, zon1_roo_solRadExc_dummyG244=7.76e-05, zon1_roo_solRadExc_dummyG245=3.723e-06, zon1_roo_solRadExc_dummyG246=4.94e-08, zon1_roo_solRadExc_dummyG247=1002.737, zon1_roo_solRadExc_dummyG248=0.012324, zon1_roo_solRadExc_dummyG249=0.02897, zon1_roo_solRadExc_dummyG250=101325, zon1_roo_solRadExc_dummyG251=0.1, zon1_roo_solRadExc_dummyG252=0.1, zon1_roo_solRadExc_dummyG253=0.8, zon1_roo_solRadExc_dummyG254=0.8, zon1_roo_solRadExc_dummyG255=0.84, zon1_roo_solRadExc_dummyG256=0.84, zon1_roo_solRadExc_dummyG257=0, zon1_roo_solRadExc_dummyG258=0, zon1_roo_solRadExc_dummyG259=3, zon1_roo_solRadExc_dummyG260=0.8, zon1_roo_solRadExc_dummyG261=0.5, zon1_roo_irRadGai_datConE262=0, zon1_roo_irRadGai_datConE263=0, zon1_roo_irRadGai_dummyCo264=0.9, zon1_roo_irRadGai_dummyCo265=0.9, zon1_roo_irRadGai_dummyCo266=0.5, zon1_roo_irRadGai_dummyCo267=0.5, zon1_roo_irRadGai_dummyCo268=3, zon1_roo_irRadGai_dummyGl269=0.003, zon1_roo_irRadGai_dummyGl270=1, zon1_roo_irRadGai_dummyGl271=0.834, zon1_roo_irRadGai_dummyGl272=0.075, zon1_roo_irRadGai_dummyGl273=0.075, zon1_roo_irRadGai_dummyGl274=0, zon1_roo_irRadGai_dummyGl275=0.84, zon1_roo_irRadGai_dummyGl276=0.84, zon1_roo_irRadGai_dummyGl277=-1, zon1_roo_irRadGai_dummyGl278=0.002873, zon1_roo_irRadGai_dummyGl279=7.76e-05, zon1_roo_irRadGai_dummyGl280=3.723e-06, zon1_roo_irRadGai_dummyGl281=4.94e-08, zon1_roo_irRadGai_dummyGl282=1002.737, zon1_roo_irRadGai_dummyGl283=0.012324, zon1_roo_irRadGai_dummyGl284=0.02897, zon1_roo_irRadGai_dummyGl285=101325, zon1_roo_irRadGai_dummyGl286=0.1, zon1_roo_irRadGai_dummyGl287=0.1, zon1_roo_irRadGai_dummyGl288=0.8, zon1_roo_irRadGai_dummyGl289=0.8, zon1_roo_irRadGai_dummyGl290=0.84, zon1_roo_irRadGai_dummyGl291=0.84, zon1_roo_irRadGai_dummyGl292=0, zon1_roo_irRadGai_dummyGl293=0, zon1_roo_irRadGai_dummyGl294=3, zon1_roo_irRadGai_dummyGl295=0.8, zon1_roo_irRadGai_dummyGl296=0.5, zon1_roo_irRadExc_datConE297=0, zon1_roo_irRadExc_datConE298=0, zon1_roo_irRadExc_dummyCo299=0.9, zon1_roo_irRadExc_dummyCo300=0.9, zon1_roo_irRadExc_dummyCo301=0.5, zon1_roo_irRadExc_dummyCo302=0.5, zon1_roo_irRadExc_dummyCo303=3, zon1_roo_irRadExc_dummyGl304=0.003, zon1_roo_irRadExc_dummyGl305=1, zon1_roo_irRadExc_dummyGl306=0.834, zon1_roo_irRadExc_dummyGl307=0.075, zon1_roo_irRadExc_dummyGl308=0.075, zon1_roo_irRadExc_dummyGl309=0, zon1_roo_irRadExc_dummyGl310=0.84, zon1_roo_irRadExc_dummyGl311=0.84, zon1_roo_irRadExc_dummyGl312=-1, zon1_roo_irRadExc_dummyGl313=0.002873, zon1_roo_irRadExc_dummyGl314=7.76e-05, zon1_roo_irRadExc_dummyGl315=3.723e-06, zon1_roo_irRadExc_dummyGl316=4.94e-08, zon1_roo_irRadExc_dummyGl317=1002.737, zon1_roo_irRadExc_dummyGl318=0.012324, zon1_roo_irRadExc_dummyGl319=0.02897, zon1_roo_irRadExc_dummyGl320=101325, zon1_roo_irRadExc_dummyGl321=0.1, zon1_roo_irRadExc_dummyGl322=0.1, zon1_roo_irRadExc_dummyGl323=0.8, zon1_roo_irRadExc_dummyGl324=0.8, zon1_roo_irRadExc_dummyGl325=0.84, zon1_roo_irRadExc_dummyGl326=0.84, zon1_roo_irRadExc_dummyGl327=0, zon1_roo_irRadExc_dummyGl328=0, zon1_roo_irRadExc_dummyGl329=3, zon1_roo_irRadExc_dummyGl330=0.8, zon1_roo_irRadExc_dummyGl331=0.5, zon1_roo_irRadExc_T0=293.15, zon1_roo_radTem_datConExt333=0, zon1_roo_radTem_datConExt334=0, zon1_roo_radTem_dummyCon_335=0.9, zon1_roo_radTem_dummyCon_336=0.9, zon1_roo_radTem_dummyCon_337=0.5, zon1_roo_radTem_dummyCon_338=0.5, zon1_roo_radTem_dummyCon_339=3, zon1_roo_radTem_dummyGlaS340=0.003, zon1_roo_radTem_dummyGlaS341=1, zon1_roo_radTem_dummyGlaS342=0.834, zon1_roo_radTem_dummyGlaS343=0.075, zon1_roo_radTem_dummyGlaS344=0.075, zon1_roo_radTem_dummyGlaS345=0, zon1_roo_radTem_dummyGlaS346=0.84, zon1_roo_radTem_dummyGlaS347=0.84, zon1_roo_radTem_dummyGlaS348=-1, zon1_roo_radTem_dummyGlaS349=0.002873, zon1_roo_radTem_dummyGlaS350=7.76e-05, zon1_roo_radTem_dummyGlaS351=3.723e-06, zon1_roo_radTem_dummyGlaS352=4.94e-08, zon1_roo_radTem_dummyGlaS353=1002.737, zon1_roo_radTem_dummyGlaS354=0.012324, zon1_roo_radTem_dummyGlaS355=0.02897, zon1_roo_radTem_dummyGlaS356=101325, zon1_roo_radTem_dummyGlaS357=0.1, zon1_roo_radTem_dummyGlaS358=0.1, zon1_roo_radTem_dummyGlaS359=0.8, zon1_roo_radTem_dummyGlaS360=0.8, zon1_roo_radTem_dummyGlaS361=0.84, zon1_roo_radTem_dummyGlaS362=0.84, zon1_roo_radTem_dummyGlaS363=0, zon1_roo_radTem_dummyGlaS364=0, zon1_roo_radTem_dummyGlaS365=3, zon1_roo_radTem_dummyGlaS366=0.8, zon1_roo_radTem_dummyGlaS367=0.5, zon1_roo_add_k1=1, zon1_roo_add_k2=1, zon1_roo_sumJFroWin_1__k=1, zon1_roo_p_start=101325, zon1_roo_T_start=293.15, zon1_roo_X_start=[0.01; 0.99], zon1_qConGai_flow_k=4, zon1_qRadGai_flow_k=6, zon1_qLatGai_flow_k=2, zon1_TSoi_1__T=283.15, zon1_sinInf_m_flow=0, zon1_sinInf_x_pTphi_p=101325, zon1_InfiltrationRate_k=0.018, zon1_souInf_m_flow=0, zon1_souInf_x_pTphi_p=101325, zon1_intLoad_table=[0; 0.1; 28800; 0.1; 28800; 1; 64800; 1; 64800; 0.1; 86400; 0.1], zon1_intLoad_verboseRead=1, zon1_intLoad_columns=2, zon1_intLoad_offset=0, zon1_intLoad_startTime=0, zon1_intLoad_timeEvents=1, weaDat_pAtm=101325, weaDat_TDryBul=293.15, weaDat_TDewPoi=283.15, weaDat_TBlaSky=273.15, weaDat_relHum=0.5, weaDat_winSpe=1, weaDat_winDir=1, weaDat_HInfHor=0, weaDat_ceiHei=20000, weaDat_totSkyCov=0.5, weaDat_opaSkyCov=0.5, weaDat_datRea_verboseRead=0, weaDat_cheTemDryBul_TMin=203.15, weaDat_cheTemDryBul_TMax=343.15, weaDat_cheTemDewPoi_TMin=203.15, weaDat_cheTemDewPoi_TMax=343.15, weaDat_add30Min_k1=1, weaDat_add30Min_k2=1, weaDat_datRea30Min_verbos407=0, weaDat_cheTemBlaSky_TMin=0, weaDat_cheTemBlaSky_TMax=343.15, rooSin_p=101325, rooSin_T=293.15, rooSin_X=[0.01; 0.99], zon2_S_=0, zon2_E_=-1.5707963267949, zon2_W_=1.5707963267949, zon2_N_=3.14159265358979, zon2_matExtWal_absIR_a=0.9, zon2_matExtWal_absIR_b=0.9, zon2_matExtWal_absSol_a=0.6, zon2_matExtWal_absSol_b=0.6, zon2_matExtWal_roughness_421=3, zon2_matFlo_absIR_a=0.9, zon2_matFlo_absIR_b=0.9, zon2_matFlo_absSol_a=0.6, zon2_matFlo_absSol_b=0.6, zon2_matFlo_roughness_a=3, zon2_roof_absIR_a=0.9, zon2_roof_absIR_b=0.9, zon2_roof_absSol_a=0.6, zon2_roof_absSol_b=0.6, zon2_roof_roughness_a=3, zon2_window600_glass_1__x=0.003175, zon2_window600_glass_1__k=1.06, zon2_window600_glass_1__t434=0.86156, zon2_window600_glass_1__r435=0.0434, zon2_window600_glass_1__r436=0.0434, zon2_window600_glass_1__t437=0, zon2_window600_glass_1__a438=0.9, zon2_window600_glass_1__a439=0.9, zon2_window600_glass_2__x=0.003175, zon2_window600_glass_2__k=1.06, zon2_window600_glass_2__t442=0.86156, zon2_window600_glass_2__r443=0.0434, zon2_window600_glass_2__r444=0.0434, zon2_window600_glass_2__t445=0, zon2_window600_glass_2__a446=0.9, zon2_window600_glass_2__a447=0.9, zon2_window600_gas_1__x=0.013, zon2_window600_gas_1__a_k=0.002873, zon2_window600_gas_1__b_k=7.76e-05, zon2_window600_gas_1__a_m451=3.723e-06, zon2_window600_gas_1__b_m452=4.94e-08, zon2_window600_gas_1__a_c=1002.737, zon2_window600_gas_1__b_c=0.012324, zon2_window600_gas_1__MM=0.02897, zon2_window600_gas_1__P0=101325, zon2_window600_shade_tauS457=0.1, zon2_window600_shade_tauS458=0.1, zon2_window600_shade_rhoS459=0.8, zon2_window600_shade_rhoS460=0.8, zon2_window600_shade_absI461=0.84, zon2_window600_shade_absI462=0.84, zon2_window600_shade_tauI463=0, zon2_window600_shade_tauI464=0, zon2_window600_UFra=3, zon2_window600_absIRFra=0.8, zon2_window600_absSolFra=0.5, zon2_soi_A=48, zon2_soi_T_a_start=283.15, zon2_soi_T_b_start=283.75, zon2_roo_datConExt_1__bou471=1, zon2_roo_datConExt_1__A=48, zon2_roo_datConExt_2__bou473=1, zon2_roo_datConExt_2__A=16.2, zon2_roo_datConExt_3__bou475=1, zon2_roo_datConExt_3__A=16.2, zon2_roo_datConExt_4__bou477=1, zon2_roo_datConExt_4__A=21.6, zon2_roo_datConExtWin_1__479=1, zon2_roo_datConExtWin_1__480=21.6, zon2_roo_datConExtWin_1__481=2, zon2_roo_datConExtWin_1__482=6, zon2_roo_datConExtWin_1__483=0.001, zon2_roo_datConExtWin_1__484=0, zon2_roo_datConExtWin_1__485=0, zon2_roo_datConExtWin_1__486=0, zon2_roo_datConExtWin_1__487=0, zon2_roo_datConExtWin_1__488=0, zon2_roo_datConPar_1__azi=0, zon2_roo_datConPar_1__bou490=1, zon2_roo_datConPar_1__A=0, zon2_roo_datConBou_1__azi=0, zon2_roo_datConBou_1__bou493=1, zon2_roo_datConBou_1__A=48, zon2_roo_surBou_1__A=0, zon2_roo_surBou_1__absIR=0.84, zon2_roo_surBou_1__absSol=0.84, zon2_roo_surBou_1__bounda498=1, zon2_roo_dummyCon_absIR_a=0.9, zon2_roo_dummyCon_absIR_b=0.9, zon2_roo_dummyCon_absSol_501=0.5, zon2_roo_dummyCon_absSol_502=0.5, zon2_roo_dummyCon_roughne503=3, zon2_roo_dummyGlaSys_glas504=0.003, zon2_roo_dummyGlaSys_glas505=1, zon2_roo_dummyGlaSys_glas506=0.834, zon2_roo_dummyGlaSys_glas507=0.075, zon2_roo_dummyGlaSys_glas508=0.075, zon2_roo_dummyGlaSys_glas509=0, zon2_roo_dummyGlaSys_glas510=0.84, zon2_roo_dummyGlaSys_glas511=0.84, zon2_roo_dummyGlaSys_gas_512=-1, zon2_roo_dummyGlaSys_gas_513=0.002873, zon2_roo_dummyGlaSys_gas_514=7.76e-05, zon2_roo_dummyGlaSys_gas_515=3.723e-06, zon2_roo_dummyGlaSys_gas_516=4.94e-08, zon2_roo_dummyGlaSys_gas_517=1002.737, zon2_roo_dummyGlaSys_gas_518=0.012324, zon2_roo_dummyGlaSys_gas_519=0.02897, zon2_roo_dummyGlaSys_gas_520=101325, zon2_roo_dummyGlaSys_shad521=0.1, zon2_roo_dummyGlaSys_shad522=0.1, zon2_roo_dummyGlaSys_shad523=0.8, zon2_roo_dummyGlaSys_shad524=0.8, zon2_roo_dummyGlaSys_shad525=0.84, zon2_roo_dummyGlaSys_shad526=0.84, zon2_roo_dummyGlaSys_shad527=0, zon2_roo_dummyGlaSys_shad528=0, zon2_roo_dummyGlaSys_UFra=3, zon2_roo_dummyGlaSys_absI530=0.8, zon2_roo_dummyGlaSys_absS531=0.5, zon2_roo_AFlo=48, zon2_roo_hRoo=2.7, zon2_roo_conExtWin_1__gla534=0, zon2_roo_conExtWin_1__win535=1, zon2_roo_conExtWin_1__win536=3, zon2_roo_conExtWin_1__win537=331.4, zon2_roo_conExtWin_1__win538=1, zon2_roo_hIntFixed=3, zon2_roo_hExtFixed=10, zon2_roo_bouConExt_HDifTi541=0.2, zon2_roo_bouConExt_HDifTi542=1, zon2_roo_bouConExt_HDifTi543=1, zon2_roo_bouConExt_HDifTi544=0.2, zon2_roo_bouConExt_HDifTi545=1, zon2_roo_bouConExt_HDifTi546=1, zon2_roo_bouConExt_HDifTi547=0.2, zon2_roo_bouConExt_HDifTi548=1, zon2_roo_bouConExt_HDifTi549=1, zon2_roo_bouConExt_HDifTi550=0.2, zon2_roo_bouConExt_HDifTi551=1, zon2_roo_bouConExt_HDifTi552=1, zon2_roo_bouConExtWin_con553=0, zon2_roo_bouConExtWin_con554=0, zon2_roo_bouConExtWin_HDi555=0.2, zon2_roo_bouConExtWin_HDi556=1, zon2_roo_bouConExtWin_HDi557=1, zon2_roo_bouConExtWin_con558=293.15, zon2_roo_air_datConExtWin559=0, zon2_roo_air_datConExtWin560=0, zon2_roo_air_dummyCon_abs561=0.9, zon2_roo_air_dummyCon_abs562=0.9, zon2_roo_air_dummyCon_abs563=0.5, zon2_roo_air_dummyCon_abs564=0.5, zon2_roo_air_dummyCon_rou565=3, zon2_roo_air_dummyGlaSys_566=0.003, zon2_roo_air_dummyGlaSys_567=1, zon2_roo_air_dummyGlaSys_568=0.834, zon2_roo_air_dummyGlaSys_569=0.075, zon2_roo_air_dummyGlaSys_570=0.075, zon2_roo_air_dummyGlaSys_571=0, zon2_roo_air_dummyGlaSys_572=0.84, zon2_roo_air_dummyGlaSys_573=0.84, zon2_roo_air_dummyGlaSys_574=-1, zon2_roo_air_dummyGlaSys_575=0.002873, zon2_roo_air_dummyGlaSys_576=7.76e-05, zon2_roo_air_dummyGlaSys_577=3.723e-06, zon2_roo_air_dummyGlaSys_578=4.94e-08, zon2_roo_air_dummyGlaSys_579=1002.737, zon2_roo_air_dummyGlaSys_580=0.012324, zon2_roo_air_dummyGlaSys_581=0.02897, zon2_roo_air_dummyGlaSys_582=101325, zon2_roo_air_dummyGlaSys_583=0.1, zon2_roo_air_dummyGlaSys_584=0.1, zon2_roo_air_dummyGlaSys_585=0.8, zon2_roo_air_dummyGlaSys_586=0.8, zon2_roo_air_dummyGlaSys_587=0.84, zon2_roo_air_dummyGlaSys_588=0.84, zon2_roo_air_dummyGlaSys_589=0, zon2_roo_air_dummyGlaSys_590=0, zon2_roo_air_dummyGlaSys_591=3, zon2_roo_air_dummyGlaSys_592=0.8, zon2_roo_air_dummyGlaSys_593=0.5, zon2_roo_solRadExc_datCon594=0, zon2_roo_solRadExc_datCon595=0, zon2_roo_solRadExc_dummyC596=0.9, zon2_roo_solRadExc_dummyC597=0.9, zon2_roo_solRadExc_dummyC598=0.5, zon2_roo_solRadExc_dummyC599=0.5, zon2_roo_solRadExc_dummyC600=3, zon2_roo_solRadExc_dummyG601=0.003, zon2_roo_solRadExc_dummyG602=1, zon2_roo_solRadExc_dummyG603=0.834, zon2_roo_solRadExc_dummyG604=0.075, zon2_roo_solRadExc_dummyG605=0.075, zon2_roo_solRadExc_dummyG606=0, zon2_roo_solRadExc_dummyG607=0.84, zon2_roo_solRadExc_dummyG608=0.84, zon2_roo_solRadExc_dummyG609=-1, zon2_roo_solRadExc_dummyG610=0.002873, zon2_roo_solRadExc_dummyG611=7.76e-05, zon2_roo_solRadExc_dummyG612=3.723e-06, zon2_roo_solRadExc_dummyG613=4.94e-08, zon2_roo_solRadExc_dummyG614=1002.737, zon2_roo_solRadExc_dummyG615=0.012324, zon2_roo_solRadExc_dummyG616=0.02897, zon2_roo_solRadExc_dummyG617=101325, zon2_roo_solRadExc_dummyG618=0.1, zon2_roo_solRadExc_dummyG619=0.1, zon2_roo_solRadExc_dummyG620=0.8, zon2_roo_solRadExc_dummyG621=0.8, zon2_roo_solRadExc_dummyG622=0.84, zon2_roo_solRadExc_dummyG623=0.84, zon2_roo_solRadExc_dummyG624=0, zon2_roo_solRadExc_dummyG625=0, zon2_roo_solRadExc_dummyG626=3, zon2_roo_solRadExc_dummyG627=0.8, zon2_roo_solRadExc_dummyG628=0.5, zon2_roo_irRadGai_datConE629=0, zon2_roo_irRadGai_datConE630=0, zon2_roo_irRadGai_dummyCo631=0.9, zon2_roo_irRadGai_dummyCo632=0.9, zon2_roo_irRadGai_dummyCo633=0.5, zon2_roo_irRadGai_dummyCo634=0.5, zon2_roo_irRadGai_dummyCo635=3, zon2_roo_irRadGai_dummyGl636=0.003, zon2_roo_irRadGai_dummyGl637=1, zon2_roo_irRadGai_dummyGl638=0.834, zon2_roo_irRadGai_dummyGl639=0.075, zon2_roo_irRadGai_dummyGl640=0.075, zon2_roo_irRadGai_dummyGl641=0, zon2_roo_irRadGai_dummyGl642=0.84, zon2_roo_irRadGai_dummyGl643=0.84, zon2_roo_irRadGai_dummyGl644=-1, zon2_roo_irRadGai_dummyGl645=0.002873, zon2_roo_irRadGai_dummyGl646=7.76e-05, zon2_roo_irRadGai_dummyGl647=3.723e-06, zon2_roo_irRadGai_dummyGl648=4.94e-08, zon2_roo_irRadGai_dummyGl649=1002.737, zon2_roo_irRadGai_dummyGl650=0.012324, zon2_roo_irRadGai_dummyGl651=0.02897, zon2_roo_irRadGai_dummyGl652=101325, zon2_roo_irRadGai_dummyGl653=0.1, zon2_roo_irRadGai_dummyGl654=0.1, zon2_roo_irRadGai_dummyGl655=0.8, zon2_roo_irRadGai_dummyGl656=0.8, zon2_roo_irRadGai_dummyGl657=0.84, zon2_roo_irRadGai_dummyGl658=0.84, zon2_roo_irRadGai_dummyGl659=0, zon2_roo_irRadGai_dummyGl660=0, zon2_roo_irRadGai_dummyGl661=3, zon2_roo_irRadGai_dummyGl662=0.8, zon2_roo_irRadGai_dummyGl663=0.5, zon2_roo_irRadExc_datConE664=0, zon2_roo_irRadExc_datConE665=0, zon2_roo_irRadExc_dummyCo666=0.9, zon2_roo_irRadExc_dummyCo667=0.9, zon2_roo_irRadExc_dummyCo668=0.5, zon2_roo_irRadExc_dummyCo669=0.5, zon2_roo_irRadExc_dummyCo670=3, zon2_roo_irRadExc_dummyGl671=0.003, zon2_roo_irRadExc_dummyGl672=1, zon2_roo_irRadExc_dummyGl673=0.834, zon2_roo_irRadExc_dummyGl674=0.075, zon2_roo_irRadExc_dummyGl675=0.075, zon2_roo_irRadExc_dummyGl676=0, zon2_roo_irRadExc_dummyGl677=0.84, zon2_roo_irRadExc_dummyGl678=0.84, zon2_roo_irRadExc_dummyGl679=-1, zon2_roo_irRadExc_dummyGl680=0.002873, zon2_roo_irRadExc_dummyGl681=7.76e-05, zon2_roo_irRadExc_dummyGl682=3.723e-06, zon2_roo_irRadExc_dummyGl683=4.94e-08, zon2_roo_irRadExc_dummyGl684=1002.737, zon2_roo_irRadExc_dummyGl685=0.012324, zon2_roo_irRadExc_dummyGl686=0.02897, zon2_roo_irRadExc_dummyGl687=101325, zon2_roo_irRadExc_dummyGl688=0.1, zon2_roo_irRadExc_dummyGl689=0.1, zon2_roo_irRadExc_dummyGl690=0.8, zon2_roo_irRadExc_dummyGl691=0.8, zon2_roo_irRadExc_dummyGl692=0.84, zon2_roo_irRadExc_dummyGl693=0.84, zon2_roo_irRadExc_dummyGl694=0, zon2_roo_irRadExc_dummyGl695=0, zon2_roo_irRadExc_dummyGl696=3, zon2_roo_irRadExc_dummyGl697=0.8, zon2_roo_irRadExc_dummyGl698=0.5, zon2_roo_irRadExc_T0=293.15, zon2_roo_radTem_datConExt700=0, zon2_roo_radTem_datConExt701=0, zon2_roo_radTem_dummyCon_702=0.9, zon2_roo_radTem_dummyCon_703=0.9, zon2_roo_radTem_dummyCon_704=0.5, zon2_roo_radTem_dummyCon_705=0.5, zon2_roo_radTem_dummyCon_706=3, zon2_roo_radTem_dummyGlaS707=0.003, zon2_roo_radTem_dummyGlaS708=1, zon2_roo_radTem_dummyGlaS709=0.834, zon2_roo_radTem_dummyGlaS710=0.075, zon2_roo_radTem_dummyGlaS711=0.075, zon2_roo_radTem_dummyGlaS712=0, zon2_roo_radTem_dummyGlaS713=0.84, zon2_roo_radTem_dummyGlaS714=0.84, zon2_roo_radTem_dummyGlaS715=-1, zon2_roo_radTem_dummyGlaS716=0.002873, zon2_roo_radTem_dummyGlaS717=7.76e-05, zon2_roo_radTem_dummyGlaS718=3.723e-06, zon2_roo_radTem_dummyGlaS719=4.94e-08, zon2_roo_radTem_dummyGlaS720=1002.737, zon2_roo_radTem_dummyGlaS721=0.012324, zon2_roo_radTem_dummyGlaS722=0.02897, zon2_roo_radTem_dummyGlaS723=101325, zon2_roo_radTem_dummyGlaS724=0.1, zon2_roo_radTem_dummyGlaS725=0.1, zon2_roo_radTem_dummyGlaS726=0.8, zon2_roo_radTem_dummyGlaS727=0.8, zon2_roo_radTem_dummyGlaS728=0.84, zon2_roo_radTem_dummyGlaS729=0.84, zon2_roo_radTem_dummyGlaS730=0, zon2_roo_radTem_dummyGlaS731=0, zon2_roo_radTem_dummyGlaS732=3, zon2_roo_radTem_dummyGlaS733=0.8, zon2_roo_radTem_dummyGlaS734=0.5, zon2_roo_add_k1=1, zon2_roo_add_k2=1, zon2_roo_sumJFroWin_1__k=1, zon2_roo_p_start=101325, zon2_roo_T_start=293.15, zon2_roo_X_start=[0.01; 0.99], zon2_qConGai_flow_k=4, zon2_qRadGai_flow_k=6, zon2_qLatGai_flow_k=2, zon2_TSoi_1__T=283.15, zon2_sinInf_m_flow=0, zon2_sinInf_x_pTphi_p=101325, zon2_InfiltrationRate_k=0.018, zon2_souInf_m_flow=0, zon2_souInf_x_pTphi_p=101325, zon2_intLoad_table=[0; 0.1; 28800; 0.1; 28800; 1; 64800; 1; 64800; 0.1; 86400; 0.1], zon2_intLoad_verboseRead=1, zon2_intLoad_columns=2, zon2_intLoad_offset=0, zon2_intLoad_startTime=0, zon2_intLoad_timeEvents=1, vav2_vav_sta_default_p=101325, vav2_vav_sta_default_T=293.15, vav2_vav_sta_default_X=[0.01; 0.99], vav2_vav_riseTime=120, vav2_vav_y_start=1, vav2_vav_filter_gain=1, vav2_vav_filter_A_ripple=0.5, vav2_vav_filter_f_min=0, vav2_vav_filter_normalize764=1, vav2_vav_filter_x_start=[0; 0], vav2_vav_filter_u_nominal=1, vav2_vav_use_deltaM=1, vav2_vav_deltaM=0.3, vav2_vav_roundDuct=0, vav2_vav_ReC=4000, vav2_vav_a=-1.51, vav2_vav_b=9.45, vav2_vav_yL=0.166666666666667, vav2_vav_yU=0.611111111111111, vav2_vav_k1=0.45, vav2_vav_l=0.0001, vav2_vav_l2=0.01, vav2_vav_deltax=0.02, vav2_vav_y_min=0.02, vav2_terHea_bal1_preDro_s780=101325, vav2_terHea_bal1_preDro_s781=293.15, vav2_terHea_bal1_preDro_s782=[0.01; 0.99], vav2_terHea_bal2_preDro_s783=300000, vav2_terHea_bal2_preDro_s784=293.15, vav2_terHea_delta=0.001, vav2_terHea_T_a1_nominal=289.85, vav2_terHea_T_a2_nominal=355.35, vav2_terHea_r_nominal=0.666666666666667, vav2_terHea_hA_n_w=0.85, vav2_terHea_hA_n_a=0.8, vav2_terHea_hA_T0_w=293.15, vav2_terHea_hA_T0_a=293.15, vav2_sinTer_X=1, vav2_sinTer_p=300000, vav2_sinTer_T=293.15, vav2_souTer_X=1, vav2_souTer_m_flow=0, vav2_souTer_T=323.15, coiSou_X=[0.01; 0.99], coiSou_T=285.15, byp_sta_default_p=101325, byp_sta_default_T=293.15, byp_sta_default_X=[0.01; 0.99], VSup2_T_start=293.15, VSup2_p_start=101325, VSup2_X_start=[0.01; 0.99], VSup1_T_start=293.15, VSup1_p_start=101325, VSup1_X_start=[0.01; 0.99], TDisVAV1_T_start=293.15, TDisVAV1_TAmb=293.15, TDisVAV1_tauHeaTra=1200, TDisVAV2_T_start=293.15, TDisVAV2_TAmb=293.15, TDisVAV2_tauHeaTra=1200, zon1_roo_conExtWin_1__win816=293.15, zon1_roo_conExtWin_1__win817=293.15, zon1_roo_conExtWin_1__win818=293.15, zon2_roo_conExtWin_1__win819=293.15, zon2_roo_conExtWin_1__win820=293.15, zon2_roo_conExtWin_1__win821=293.15}
      mask prompts: vav1_vav_sta_default_p "vav1.vav.sta_default.p"; vav1_vav_sta_default_T "vav1.vav.sta_default.T"; vav1_vav_sta_default_X "vav1.vav.sta_default.X"; vav1_vav_riseTime "vav1.vav.riseTime"; vav1_vav_y_start "vav1.vav.y_start"; vav1_vav_filter_gain "vav1.vav.filter.gain"; vav1_vav_filter_A_ripple "vav1.vav.filter.A_ripple"; vav1_vav_filter_f_min "vav1.vav.filter.f_min"; vav1_vav_filter_normalize10 "vav1.vav.filter.normalized"; vav1_vav_filter_x_start "vav1.vav.filter.x_start"; vav1_vav_filter_u_nominal "vav1.vav.filter.u_nominal"; vav1_vav_use_deltaM "vav1.vav.use_deltaM"; vav1_vav_deltaM "vav1.vav.deltaM"; vav1_vav_roundDuct "vav1.vav.roundDuct"; vav1_vav_ReC "vav1.vav.ReC"; vav1_vav_a "vav1.vav.a"; vav1_vav_b "vav1.vav.b"; vav1_vav_yL "vav1.vav.yL"; vav1_vav_yU "vav1.vav.yU"; vav1_vav_k1 "vav1.vav.k1"; vav1_vav_l "vav1.vav.l"; vav1_vav_l2 "vav1.vav.l2"; vav1_vav_deltax "vav1.vav.deltax"; vav1_vav_y_min "vav1.vav.y_min"; vav1_terHea_bal1_preDro_s26 "vav1.terHea.bal1.preDro.sta_default.p"; vav1_terHea_bal1_preDro_s27 "vav1.terHea.bal1.preDro.sta_default.T"; vav1_terHea_bal1_preDro_s28 "vav1.terHea.bal1.preDro.sta_default.X"; vav1_terHea_bal2_preDro_s29 "vav1.terHea.bal2.preDro.sta_default.p"; vav1_terHea_bal2_preDro_s30 "vav1.terHea.bal2.preDro.sta_default.T"; vav1_terHea_delta "vav1.terHea.delta"; vav1_terHea_T_a1_nominal "vav1.terHea.T_a1_nominal"; vav1_terHea_T_a2_nominal "vav1.terHea.T_a2_nominal"; vav1_terHea_r_nominal "vav1.terHea.r_nominal"; vav1_terHea_hA_n_w "vav1.terHea.hA.n_w"; vav1_terHea_hA_n_a "vav1.terHea.hA.n_a"; vav1_terHea_hA_T0_w "vav1.terHea.hA.T0_w"; vav1_terHea_hA_T0_a "vav1.terHea.hA.T0_a"; vav1_sinTer_X "vav1.sinTer.X"; vav1_sinTer_p "vav1.sinTer.p"; vav1_sinTer_T "vav1.sinTer.T"; vav1_souTer_X "vav1.souTer.X"; vav1_souTer_m_flow "vav1.souTer.m_flow"; vav1_souTer_T "vav1.souTer.T"; zer_k "zer.k"; zon1_S_ "zon1.S_"; zon1_E_ "zon1.E_"; zon1_W_ "zon1.W_"; zon1_N_ "zon1.N_"; zon1_matExtWal_absIR_a "zon1.matExtWal.absIR_a"; zon1_matExtWal_absIR_b "zon1.matExtWal.absIR_b"; zon1_matExtWal_absSol_a "zon1.matExtWal.absSol_a"; zon1_matExtWal_absSol_b "zon1.matExtWal.absSol_b"; zon1_matExtWal_roughness_54 "zon1.matExtWal.roughness_a"; zon1_matFlo_absIR_a "zon1.matFlo.absIR_a"; zon1_matFlo_absIR_b "zon1.matFlo.absIR_b"; zon1_matFlo_absSol_a "zon1.matFlo.absSol_a"; zon1_matFlo_absSol_b "zon1.matFlo.absSol_b"; zon1_matFlo_roughness_a "zon1.matFlo.roughness_a"; zon1_roof_absIR_a "zon1.roof.absIR_a"; zon1_roof_absIR_b "zon1.roof.absIR_b"; zon1_roof_absSol_a "zon1.roof.absSol_a"; zon1_roof_absSol_b "zon1.roof.absSol_b"; zon1_roof_roughness_a "zon1.roof.roughness_a"; zon1_window600_glass_1__x "zon1.window600.glass[1].x"; zon1_window600_glass_1__k "zon1.window600.glass[1].k"; zon1_window600_glass_1__t67 "zon1.window600.glass[1].tauSol"; zon1_window600_glass_1__r68 "zon1.window600.glass[1].rhoSol_a"; zon1_window600_glass_1__r69 "zon1.window600.glass[1].rhoSol_b"; zon1_window600_glass_1__t70 "zon1.window600.glass[1].tauIR"; zon1_window600_glass_1__a71 "zon1.window600.glass[1].absIR_a"; zon1_window600_glass_1__a72 "zon1.window600.glass[1].absIR_b"; zon1_window600_glass_2__x "zon1.window600.glass[2].x"; zon1_window600_glass_2__k "zon1.window600.glass[2].k"; zon1_window600_glass_2__t75 "zon1.window600.glass[2].tauSol"; zon1_window600_glass_2__r76 "zon1.window600.glass[2].rhoSol_a"; zon1_window600_glass_2__r77 "zon1.window600.glass[2].rhoSol_b"; zon1_window600_glass_2__t78 "zon1.window600.glass[2].tauIR"; zon1_window600_glass_2__a79 "zon1.window600.glass[2].absIR_a"; zon1_window600_glass_2__a80 "zon1.window600.glass[2].absIR_b"; zon1_window600_gas_1__x "zon1.window600.gas[1].x"; zon1_window600_gas_1__a_k "zon1.window600.gas[1].a_k"; zon1_window600_gas_1__b_k "zon1.window600.gas[1].b_k"; zon1_window600_gas_1__a_m84 "zon1.window600.gas[1].a_mu"; zon1_window600_gas_1__b_m85 "zon1.window600.gas[1].b_mu"; zon1_window600_gas_1__a_c "zon1.window600.gas[1].a_c"; zon1_window600_gas_1__b_c "zon1.window600.gas[1].b_c"; zon1_window600_gas_1__MM "zon1.window600.gas[1].MM"; zon1_window600_gas_1__P0 "zon1.window600.gas[1].P0"; zon1_window600_shade_tauS90 "zon1.window600.shade.tauSol_a"; zon1_window600_shade_tauS91 "zon1.window600.shade.tauSol_b"; zon1_window600_shade_rhoS92 "zon1.window600.shade.rhoSol_a"; zon1_window600_shade_rhoS93 "zon1.window600.shade.rhoSol_b"; zon1_window600_shade_absI94 "zon1.window600.shade.absIR_a"; zon1_window600_shade_absI95 "zon1.window600.shade.absIR_b"; zon1_window600_shade_tauI96 "zon1.window600.shade.tauIR_a"; zon1_window600_shade_tauI97 "zon1.window600.shade.tauIR_b"; zon1_window600_UFra "zon1.window600.UFra"; zon1_window600_absIRFra "zon1.window600.absIRFra"; zon1_window600_absSolFra "zon1.window600.absSolFra"; zon1_soi_A "zon1.soi.A"; zon1_soi_T_a_start "zon1.soi.T_a_start"; zon1_soi_T_b_start "zon1.soi.T_b_start"; zon1_roo_datConExt_1__bou104 "zon1.roo.datConExt[1].boundaryCondition"; zon1_roo_datConExt_1__A "zon1.roo.datConExt[1].A"; zon1_roo_datConExt_2__bou106 "zon1.roo.datConExt[2].boundaryCondition"; zon1_roo_datConExt_2__A "zon1.roo.datConExt[2].A"; zon1_roo_datConExt_3__bou108 "zon1.roo.datConExt[3].boundaryCondition"; zon1_roo_datConExt_3__A "zon1.roo.datConExt[3].A"; zon1_roo_datConExt_4__bou110 "zon1.roo.datConExt[4].boundaryCondition"; zon1_roo_datConExt_4__A "zon1.roo.datConExt[4].A"; zon1_roo_datConExtWin_1__112 "zon1.roo.datConExtWin[1].boundaryCondition"; zon1_roo_datConExtWin_1__113 "zon1.roo.datConExtWin[1].A"; zon1_roo_datConExtWin_1__114 "zon1.roo.datConExtWin[1].hWin"; zon1_roo_datConExtWin_1__115 "zon1.roo.datConExtWin[1].wWin"; zon1_roo_datConExtWin_1__116 "zon1.roo.datConExtWin[1].fFra"; zon1_roo_datConExtWin_1__117 "zon1.roo.datConExtWin[1].ove.wL"; zon1_roo_datConExtWin_1__118 "zon1.roo.datConExtWin[1].ove.wR"; zon1_roo_datConExtWin_1__119 "zon1.roo.datConExtWin[1].ove.gap"; zon1_roo_datConExtWin_1__120 "zon1.roo.datConExtWin[1].sidFin.h"; zon1_roo_datConExtWin_1__121 "zon1.roo.datConExtWin[1].sidFin.gap"; zon1_roo_datConPar_1__azi "zon1.roo.datConPar[1].azi"; zon1_roo_datConPar_1__bou123 "zon1.roo.datConPar[1].boundaryCondition"; zon1_roo_datConPar_1__A "zon1.roo.datConPar[1].A"; zon1_roo_datConBou_1__azi "zon1.roo.datConBou[1].azi"; zon1_roo_datConBou_1__bou126 "zon1.roo.datConBou[1].boundaryCondition"; zon1_roo_datConBou_1__A "zon1.roo.datConBou[1].A"; zon1_roo_surBou_1__A "zon1.roo.surBou[1].A"; zon1_roo_surBou_1__absIR "zon1.roo.surBou[1].absIR"; zon1_roo_surBou_1__absSol "zon1.roo.surBou[1].absSol"; zon1_roo_surBou_1__bounda131 "zon1.roo.surBou[1].boundaryCondition"; zon1_roo_dummyCon_absIR_a "zon1.roo.dummyCon.absIR_a"; zon1_roo_dummyCon_absIR_b "zon1.roo.dummyCon.absIR_b"; zon1_roo_dummyCon_absSol_134 "zon1.roo.dummyCon.absSol_a"; zon1_roo_dummyCon_absSol_135 "zon1.roo.dummyCon.absSol_b"; zon1_roo_dummyCon_roughne136 "zon1.roo.dummyCon.roughness_a"; zon1_roo_dummyGlaSys_glas137 "zon1.roo.dummyGlaSys.glass[1].x"; zon1_roo_dummyGlaSys_glas138 "zon1.roo.dummyGlaSys.glass[1].k"; zon1_roo_dummyGlaSys_glas139 "zon1.roo.dummyGlaSys.glass[1].tauSol"; zon1_roo_dummyGlaSys_glas140 "zon1.roo.dummyGlaSys.glass[1].rhoSol_a"; zon1_roo_dummyGlaSys_glas141 "zon1.roo.dummyGlaSys.glass[1].rhoSol_b"; zon1_roo_dummyGlaSys_glas142 "zon1.roo.dummyGlaSys.glass[1].tauIR"; zon1_roo_dummyGlaSys_glas143 "zon1.roo.dummyGlaSys.glass[1].absIR_a"; zon1_roo_dummyGlaSys_glas144 "zon1.roo.dummyGlaSys.glass[1].absIR_b"; zon1_roo_dummyGlaSys_gas_145 "zon1.roo.dummyGlaSys.gas[1].x"; zon1_roo_dummyGlaSys_gas_146 "zon1.roo.dummyGlaSys.gas[1].a_k"; zon1_roo_dummyGlaSys_gas_147 "zon1.roo.dummyGlaSys.gas[1].b_k"; zon1_roo_dummyGlaSys_gas_148 "zon1.roo.dummyGlaSys.gas[1].a_mu"; zon1_roo_dummyGlaSys_gas_149 "zon1.roo.dummyGlaSys.gas[1].b_mu"; zon1_roo_dummyGlaSys_gas_150 "zon1.roo.dummyGlaSys.gas[1].a_c"; zon1_roo_dummyGlaSys_gas_151 "zon1.roo.dummyGlaSys.gas[1].b_c"; zon1_roo_dummyGlaSys_gas_152 "zon1.roo.dummyGlaSys.gas[1].MM"; zon1_roo_dummyGlaSys_gas_153 "zon1.roo.dummyGlaSys.gas[1].P0"; zon1_roo_dummyGlaSys_shad154 "zon1.roo.dummyGlaSys.shade.tauSol_a"; zon1_roo_dummyGlaSys_shad155 "zon1.roo.dummyGlaSys.shade.tauSol_b"; zon1_roo_dummyGlaSys_shad156 "zon1.roo.dummyGlaSys.shade.rhoSol_a"; zon1_roo_dummyGlaSys_shad157 "zon1.roo.dummyGlaSys.shade.rhoSol_b"; zon1_roo_dummyGlaSys_shad158 "zon1.roo.dummyGlaSys.shade.absIR_a"; zon1_roo_dummyGlaSys_shad159 "zon1.roo.dummyGlaSys.shade.absIR_b"; zon1_roo_dummyGlaSys_shad160 "zon1.roo.dummyGlaSys.shade.tauIR_a"; zon1_roo_dummyGlaSys_shad161 "zon1.roo.dummyGlaSys.shade.tauIR_b"; zon1_roo_dummyGlaSys_UFra "zon1.roo.dummyGlaSys.UFra"; zon1_roo_dummyGlaSys_absI163 "zon1.roo.dummyGlaSys.absIRFra"; zon1_roo_dummyGlaSys_absS164 "zon1.roo.dummyGlaSys.absSolFra"; zon1_roo_AFlo "zon1.roo.AFlo"; zon1_roo_hRoo "zon1.roo.hRoo"; zon1_roo_conExtWin_1__gla167 "zon1.roo.conExtWin[1].glaSys.haveControllableWindow"; zon1_roo_conExtWin_1__win168 "zon1.roo.conExtWin[1].win.matGla.k"; zon1_roo_conExtWin_1__win169 "zon1.roo.conExtWin[1].win.matGla.nStaRef"; zon1_roo_conExtWin_1__win170 "zon1.roo.conExtWin[1].win.matGla.piRef"; zon1_roo_conExtWin_1__win171 "zon1.roo.conExtWin[1].win.matGla.nStaReal"; zon1_roo_hIntFixed "zon1.roo.hIntFixed"; zon1_roo_hExtFixed "zon1.roo.hExtFixed"; zon1_roo_bouConExt_HDifTi174 "zon1.roo.bouConExt.HDifTil[1].rho"; zon1_roo_bouConExt_HDifTi175 "zon1.roo.bouConExt.HDifTil[1].add.k1"; zon1_roo_bouConExt_HDifTi176 "zon1.roo.bouConExt.HDifTil[1].add.k2"; zon1_roo_bouConExt_HDifTi177 "zon1.roo.bouConExt.HDifTil[2].rho"; zon1_roo_bouConExt_HDifTi178 "zon1.roo.bouConExt.HDifTil[2].add.k1"; zon1_roo_bouConExt_HDifTi179 "zon1.roo.bouConExt.HDifTil[2].add.k2"; zon1_roo_bouConExt_HDifTi180 "zon1.roo.bouConExt.HDifTil[3].rho"; zon1_roo_bouConExt_HDifTi181 "zon1.roo.bouConExt.HDifTil[3].add.k1"; zon1_roo_bouConExt_HDifTi182 "zon1.roo.bouConExt.HDifTil[3].add.k2"; zon1_roo_bouConExt_HDifTi183 "zon1.roo.bouConExt.HDifTil[4].rho"; zon1_roo_bouConExt_HDifTi184 "zon1.roo.bouConExt.HDifTil[4].add.k1"; zon1_roo_bouConExt_HDifTi185 "zon1.roo.bouConExt.HDifTil[4].add.k2"; zon1_roo_bouConExtWin_con186 "zon1.roo.bouConExtWin.conPar[1].ove.dep"; zon1_roo_bouConExtWin_con187 "zon1.roo.bouConExtWin.conPar[1].sidFin.dep"; zon1_roo_bouConExtWin_HDi188 "zon1.roo.bouConExtWin.HDifTil[1].rho"; zon1_roo_bouConExtWin_HDi189 "zon1.roo.bouConExtWin.HDifTil[1].add.k1"; zon1_roo_bouConExtWin_HDi190 "zon1.roo.bouConExtWin.HDifTil[1].add.k2"; zon1_roo_bouConExtWin_con191 "zon1.roo.bouConExtWin.conExtWin[1].radOut.T0"; zon1_roo_air_datConExtWin192 "zon1.roo.air.datConExtWin[1].ove.dep"; zon1_roo_air_datConExtWin193 "zon1.roo.air.datConExtWin[1].sidFin.dep"; zon1_roo_air_dummyCon_abs194 "zon1.roo.air.dummyCon.absIR_a"; zon1_roo_air_dummyCon_abs195 "zon1.roo.air.dummyCon.absIR_b"; zon1_roo_air_dummyCon_abs196 "zon1.roo.air.dummyCon.absSol_a"; zon1_roo_air_dummyCon_abs197 "zon1.roo.air.dummyCon.absSol_b"; zon1_roo_air_dummyCon_rou198 "zon1.roo.air.dummyCon.roughness_a"; zon1_roo_air_dummyGlaSys_199 "zon1.roo.air.dummyGlaSys.glass[1].x"; zon1_roo_air_dummyGlaSys_200 "zon1.roo.air.dummyGlaSys.glass[1].k"; zon1_roo_air_dummyGlaSys_201 "zon1.roo.air.dummyGlaSys.glass[1].tauSol"; zon1_roo_air_dummyGlaSys_202 "zon1.roo.air.dummyGlaSys.glass[1].rhoSol_a"; zon1_roo_air_dummyGlaSys_203 "zon1.roo.air.dummyGlaSys.glass[1].rhoSol_b"; zon1_roo_air_dummyGlaSys_204 "zon1.roo.air.dummyGlaSys.glass[1].tauIR"; zon1_roo_air_dummyGlaSys_205 "zon1.roo.air.dummyGlaSys.glass[1].absIR_a"; zon1_roo_air_dummyGlaSys_206 "zon1.roo.air.dummyGlaSys.glass[1].absIR_b"; zon1_roo_air_dummyGlaSys_207 "zon1.roo.air.dummyGlaSys.gas[1].x"; zon1_roo_air_dummyGlaSys_208 "zon1.roo.air.dummyGlaSys.gas[1].a_k"; zon1_roo_air_dummyGlaSys_209 "zon1.roo.air.dummyGlaSys.gas[1].b_k"; zon1_roo_air_dummyGlaSys_210 "zon1.roo.air.dummyGlaSys.gas[1].a_mu"; zon1_roo_air_dummyGlaSys_211 "zon1.roo.air.dummyGlaSys.gas[1].b_mu"; zon1_roo_air_dummyGlaSys_212 "zon1.roo.air.dummyGlaSys.gas[1].a_c"; zon1_roo_air_dummyGlaSys_213 "zon1.roo.air.dummyGlaSys.gas[1].b_c"; zon1_roo_air_dummyGlaSys_214 "zon1.roo.air.dummyGlaSys.gas[1].MM"; zon1_roo_air_dummyGlaSys_215 "zon1.roo.air.dummyGlaSys.gas[1].P0"; zon1_roo_air_dummyGlaSys_216 "zon1.roo.air.dummyGlaSys.shade.tauSol_a"; zon1_roo_air_dummyGlaSys_217 "zon1.roo.air.dummyGlaSys.shade.tauSol_b"; zon1_roo_air_dummyGlaSys_218 "zon1.roo.air.dummyGlaSys.shade.rhoSol_a"; zon1_roo_air_dummyGlaSys_219 "zon1.roo.air.dummyGlaSys.shade.rhoSol_b"; zon1_roo_air_dummyGlaSys_220 "zon1.roo.air.dummyGlaSys.shade.absIR_a"; zon1_roo_air_dummyGlaSys_221 "zon1.roo.air.dummyGlaSys.shade.absIR_b"; zon1_roo_air_dummyGlaSys_222 "zon1.roo.air.dummyGlaSys.shade.tauIR_a"; zon1_roo_air_dummyGlaSys_223 "zon1.roo.air.dummyGlaSys.shade.tauIR_b"; zon1_roo_air_dummyGlaSys_224 "zon1.roo.air.dummyGlaSys.UFra"; zon1_roo_air_dummyGlaSys_225 "zon1.roo.air.dummyGlaSys.absIRFra"; zon1_roo_air_dummyGlaSys_226 "zon1.roo.air.dummyGlaSys.absSolFra"; zon1_roo_solRadExc_datCon227 "zon1.roo.solRadExc.datConExtWin[1].ove.dep"; zon1_roo_solRadExc_datCon228 "zon1.roo.solRadExc.datConExtWin[1].sidFin.dep"; zon1_roo_solRadExc_dummyC229 "zon1.roo.solRadExc.dummyCon.absIR_a"; zon1_roo_solRadExc_dummyC230 "zon1.roo.solRadExc.dummyCon.absIR_b"; zon1_roo_solRadExc_dummyC231 "zon1.roo.solRadExc.dummyCon.absSol_a"; zon1_roo_solRadExc_dummyC232 "zon1.roo.solRadExc.dummyCon.absSol_b"; zon1_roo_solRadExc_dummyC233 "zon1.roo.solRadExc.dummyCon.roughness_a"; zon1_roo_solRadExc_dummyG234 "zon1.roo.solRadExc.dummyGlaSys.glass[1].x"; zon1_roo_solRadExc_dummyG235 "zon1.roo.solRadExc.dummyGlaSys.glass[1].k"; zon1_roo_solRadExc_dummyG236 "zon1.roo.solRadExc.dummyGlaSys.glass[1].tauSol"; zon1_roo_solRadExc_dummyG237 "zon1.roo.solRadExc.dummyGlaSys.glass[1].rhoSol_a"; zon1_roo_solRadExc_dummyG238 "zon1.roo.solRadExc.dummyGlaSys.glass[1].rhoSol_b"; zon1_roo_solRadExc_dummyG239 "zon1.roo.solRadExc.dummyGlaSys.glass[1].tauIR"; zon1_roo_solRadExc_dummyG240 "zon1.roo.solRadExc.dummyGlaSys.glass[1].absIR_a"; zon1_roo_solRadExc_dummyG241 "zon1.roo.solRadExc.dummyGlaSys.glass[1].absIR_b"; zon1_roo_solRadExc_dummyG242 "zon1.roo.solRadExc.dummyGlaSys.gas[1].x"; zon1_roo_solRadExc_dummyG243 "zon1.roo.solRadExc.dummyGlaSys.gas[1].a_k"; zon1_roo_solRadExc_dummyG244 "zon1.roo.solRadExc.dummyGlaSys.gas[1].b_k"; zon1_roo_solRadExc_dummyG245 "zon1.roo.solRadExc.dummyGlaSys.gas[1].a_mu"; zon1_roo_solRadExc_dummyG246 "zon1.roo.solRadExc.dummyGlaSys.gas[1].b_mu"; zon1_roo_solRadExc_dummyG247 "zon1.roo.solRadExc.dummyGlaSys.gas[1].a_c"; zon1_roo_solRadExc_dummyG248 "zon1.roo.solRadExc.dummyGlaSys.gas[1].b_c"; zon1_roo_solRadExc_dummyG249 "zon1.roo.solRadExc.dummyGlaSys.gas[1].MM"; zon1_roo_solRadExc_dummyG250 "zon1.roo.solRadExc.dummyGlaSys.gas[1].P0"; zon1_roo_solRadExc_dummyG251 "zon1.roo.solRadExc.dummyGlaSys.shade.tauSol_a"; zon1_roo_solRadExc_dummyG252 "zon1.roo.solRadExc.dummyGlaSys.shade.tauSol_b"; zon1_roo_solRadExc_dummyG253 "zon1.roo.solRadExc.dummyGlaSys.shade.rhoSol_a"; zon1_roo_solRadExc_dummyG254 "zon1.roo.solRadExc.dummyGlaSys.shade.rhoSol_b"; zon1_roo_solRadExc_dummyG255 "zon1.roo.solRadExc.dummyGlaSys.shade.absIR_a"; zon1_roo_solRadExc_dummyG256 "zon1.roo.solRadExc.dummyGlaSys.shade.absIR_b"; zon1_roo_solRadExc_dummyG257 "zon1.roo.solRadExc.dummyGlaSys.shade.tauIR_a"; zon1_roo_solRadExc_dummyG258 "zon1.roo.solRadExc.dummyGlaSys.shade.tauIR_b"; zon1_roo_solRadExc_dummyG259 "zon1.roo.solRadExc.dummyGlaSys.UFra"; zon1_roo_solRadExc_dummyG260 "zon1.roo.solRadExc.dummyGlaSys.absIRFra"; zon1_roo_solRadExc_dummyG261 "zon1.roo.solRadExc.dummyGlaSys.absSolFra"; zon1_roo_irRadGai_datConE262 "zon1.roo.irRadGai.datConExtWin[1].ove.dep"; zon1_roo_irRadGai_datConE263 "zon1.roo.irRadGai.datConExtWin[1].sidFin.dep"; zon1_roo_irRadGai_dummyCo264 "zon1.roo.irRadGai.dummyCon.absIR_a"; zon1_roo_irRadGai_dummyCo265 "zon1.roo.irRadGai.dummyCon.absIR_b"; zon1_roo_irRadGai_dummyCo266 "zon1.roo.irRadGai.dummyCon.absSol_a"; zon1_roo_irRadGai_dummyCo267 "zon1.roo.irRadGai.dummyCon.absSol_b"; zon1_roo_irRadGai_dummyCo268 "zon1.roo.irRadGai.dummyCon.roughness_a"; zon1_roo_irRadGai_dummyGl269 "zon1.roo.irRadGai.dummyGlaSys.glass[1].x"; zon1_roo_irRadGai_dummyGl270 "zon1.roo.irRadGai.dummyGlaSys.glass[1].k"; zon1_roo_irRadGai_dummyGl271 "zon1.roo.irRadGai.dummyGlaSys.glass[1].tauSol"; zon1_roo_irRadGai_dummyGl272 "zon1.roo.irRadGai.dummyGlaSys.glass[1].rhoSol_a"; zon1_roo_irRadGai_dummyGl273 "zon1.roo.irRadGai.dummyGlaSys.glass[1].rhoSol_b"; zon1_roo_irRadGai_dummyGl274 "zon1.roo.irRadGai.dummyGlaSys.glass[1].tauIR"; zon1_roo_irRadGai_dummyGl275 "zon1.roo.irRadGai.dummyGlaSys.glass[1].absIR_a"; zon1_roo_irRadGai_dummyGl276 "zon1.roo.irRadGai.dummyGlaSys.glass[1].absIR_b"; zon1_roo_irRadGai_dummyGl277 "zon1.roo.irRadGai.dummyGlaSys.gas[1].x"; zon1_roo_irRadGai_dummyGl278 "zon1.roo.irRadGai.dummyGlaSys.gas[1].a_k"; zon1_roo_irRadGai_dummyGl279 "zon1.roo.irRadGai.dummyGlaSys.gas[1].b_k"; zon1_roo_irRadGai_dummyGl280 "zon1.roo.irRadGai.dummyGlaSys.gas[1].a_mu"; zon1_roo_irRadGai_dummyGl281 "zon1.roo.irRadGai.dummyGlaSys.gas[1].b_mu"; zon1_roo_irRadGai_dummyGl282 "zon1.roo.irRadGai.dummyGlaSys.gas[1].a_c"; zon1_roo_irRadGai_dummyGl283 "zon1.roo.irRadGai.dummyGlaSys.gas[1].b_c"; zon1_roo_irRadGai_dummyGl284 "zon1.roo.irRadGai.dummyGlaSys.gas[1].MM"; zon1_roo_irRadGai_dummyGl285 "zon1.roo.irRadGai.dummyGlaSys.gas[1].P0"; zon1_roo_irRadGai_dummyGl286 "zon1.roo.irRadGai.dummyGlaSys.shade.tauSol_a"; zon1_roo_irRadGai_dummyGl287 "zon1.roo.irRadGai.dummyGlaSys.shade.tauSol_b"; zon1_roo_irRadGai_dummyGl288 "zon1.roo.irRadGai.dummyGlaSys.shade.rhoSol_a"; zon1_roo_irRadGai_dummyGl289 "zon1.roo.irRadGai.dummyGlaSys.shade.rhoSol_b"; zon1_roo_irRadGai_dummyGl290 "zon1.roo.irRadGai.dummyGlaSys.shade.absIR_a"; zon1_roo_irRadGai_dummyGl291 "zon1.roo.irRadGai.dummyGlaSys.shade.absIR_b"; zon1_roo_irRadGai_dummyGl292 "zon1.roo.irRadGai.dummyGlaSys.shade.tauIR_a"; zon1_roo_irRadGai_dummyGl293 "zon1.roo.irRadGai.dummyGlaSys.shade.tauIR_b"; zon1_roo_irRadGai_dummyGl294 "zon1.roo.irRadGai.dummyGlaSys.UFra"; zon1_roo_irRadGai_dummyGl295 "zon1.roo.irRadGai.dummyGlaSys.absIRFra"; zon1_roo_irRadGai_dummyGl296 "zon1.roo.irRadGai.dummyGlaSys.absSolFra"; zon1_roo_irRadExc_datConE297 "zon1.roo.irRadExc.datConExtWin[1].ove.dep"; zon1_roo_irRadExc_datConE298 "zon1.roo.irRadExc.datConExtWin[1].sidFin.dep"; zon1_roo_irRadExc_dummyCo299 "zon1.roo.irRadExc.dummyCon.absIR_a"; zon1_roo_irRadExc_dummyCo300 "zon1.roo.irRadExc.dummyCon.absIR_b"; zon1_roo_irRadExc_dummyCo301 "zon1.roo.irRadExc.dummyCon.absSol_a"; zon1_roo_irRadExc_dummyCo302 "zon1.roo.irRadExc.dummyCon.absSol_b"; zon1_roo_irRadExc_dummyCo303 "zon1.roo.irRadExc.dummyCon.roughness_a"; zon1_roo_irRadExc_dummyGl304 "zon1.roo.irRadExc.dummyGlaSys.glass[1].x"; zon1_roo_irRadExc_dummyGl305 "zon1.roo.irRadExc.dummyGlaSys.glass[1].k"; zon1_roo_irRadExc_dummyGl306 "zon1.roo.irRadExc.dummyGlaSys.glass[1].tauSol"; zon1_roo_irRadExc_dummyGl307 "zon1.roo.irRadExc.dummyGlaSys.glass[1].rhoSol_a"; zon1_roo_irRadExc_dummyGl308 "zon1.roo.irRadExc.dummyGlaSys.glass[1].rhoSol_b"; zon1_roo_irRadExc_dummyGl309 "zon1.roo.irRadExc.dummyGlaSys.glass[1].tauIR"; zon1_roo_irRadExc_dummyGl310 "zon1.roo.irRadExc.dummyGlaSys.glass[1].absIR_a"; zon1_roo_irRadExc_dummyGl311 "zon1.roo.irRadExc.dummyGlaSys.glass[1].absIR_b"; zon1_roo_irRadExc_dummyGl312 "zon1.roo.irRadExc.dummyGlaSys.gas[1].x"; zon1_roo_irRadExc_dummyGl313 "zon1.roo.irRadExc.dummyGlaSys.gas[1].a_k"; zon1_roo_irRadExc_dummyGl314 "zon1.roo.irRadExc.dummyGlaSys.gas[1].b_k"; zon1_roo_irRadExc_dummyGl315 "zon1.roo.irRadExc.dummyGlaSys.gas[1].a_mu"; zon1_roo_irRadExc_dummyGl316 "zon1.roo.irRadExc.dummyGlaSys.gas[1].b_mu"; zon1_roo_irRadExc_dummyGl317 "zon1.roo.irRadExc.dummyGlaSys.gas[1].a_c"; zon1_roo_irRadExc_dummyGl318 "zon1.roo.irRadExc.dummyGlaSys.gas[1].b_c"; zon1_roo_irRadExc_dummyGl319 "zon1.roo.irRadExc.dummyGlaSys.gas[1].MM"; zon1_roo_irRadExc_dummyGl320 "zon1.roo.irRadExc.dummyGlaSys.gas[1].P0"; zon1_roo_irRadExc_dummyGl321 "zon1.roo.irRadExc.dummyGlaSys.shade.tauSol_a"; zon1_roo_irRadExc_dummyGl322 "zon1.roo.irRadExc.dummyGlaSys.shade.tauSol_b"; zon1_roo_irRadExc_dummyGl323 "zon1.roo.irRadExc.dummyGlaSys.shade.rhoSol_a"; zon1_roo_irRadExc_dummyGl324 "zon1.roo.irRadExc.dummyGlaSys.shade.rhoSol_b"; zon1_roo_irRadExc_dummyGl325 "zon1.roo.irRadExc.dummyGlaSys.shade.absIR_a"; zon1_roo_irRadExc_dummyGl326 "zon1.roo.irRadExc.dummyGlaSys.shade.absIR_b"; zon1_roo_irRadExc_dummyGl327 "zon1.roo.irRadExc.dummyGlaSys.shade.tauIR_a"; zon1_roo_irRadExc_dummyGl328 "zon1.roo.irRadExc.dummyGlaSys.shade.tauIR_b"; zon1_roo_irRadExc_dummyGl329 "zon1.roo.irRadExc.dummyGlaSys.UFra"; zon1_roo_irRadExc_dummyGl330 "zon1.roo.irRadExc.dummyGlaSys.absIRFra"; zon1_roo_irRadExc_dummyGl331 "zon1.roo.irRadExc.dummyGlaSys.absSolFra"; zon1_roo_irRadExc_T0 "zon1.roo.irRadExc.T0"; zon1_roo_radTem_datConExt333 "zon1.roo.radTem.datConExtWin[1].ove.dep"; zon1_roo_radTem_datConExt334 "zon1.roo.radTem.datConExtWin[1].sidFin.dep"; zon1_roo_radTem_dummyCon_335 "zon1.roo.radTem.dummyCon.absIR_a"; zon1_roo_radTem_dummyCon_336 "zon1.roo.radTem.dummyCon.absIR_b"; zon1_roo_radTem_dummyCon_337 "zon1.roo.radTem.dummyCon.absSol_a"; zon1_roo_radTem_dummyCon_338 "zon1.roo.radTem.dummyCon.absSol_b"; zon1_roo_radTem_dummyCon_339 "zon1.roo.radTem.dummyCon.roughness_a"; zon1_roo_radTem_dummyGlaS340 "zon1.roo.radTem.dummyGlaSys.glass[1].x"; zon1_roo_radTem_dummyGlaS341 "zon1.roo.radTem.dummyGlaSys.glass[1].k"; zon1_roo_radTem_dummyGlaS342 "zon1.roo.radTem.dummyGlaSys.glass[1].tauSol"; zon1_roo_radTem_dummyGlaS343 "zon1.roo.radTem.dummyGlaSys.glass[1].rhoSol_a"; zon1_roo_radTem_dummyGlaS344 "zon1.roo.radTem.dummyGlaSys.glass[1].rhoSol_b"; zon1_roo_radTem_dummyGlaS345 "zon1.roo.radTem.dummyGlaSys.glass[1].tauIR"; zon1_roo_radTem_dummyGlaS346 "zon1.roo.radTem.dummyGlaSys.glass[1].absIR_a"; zon1_roo_radTem_dummyGlaS347 "zon1.roo.radTem.dummyGlaSys.glass[1].absIR_b"; zon1_roo_radTem_dummyGlaS348 "zon1.roo.radTem.dummyGlaSys.gas[1].x"; zon1_roo_radTem_dummyGlaS349 "zon1.roo.radTem.dummyGlaSys.gas[1].a_k"; zon1_roo_radTem_dummyGlaS350 "zon1.roo.radTem.dummyGlaSys.gas[1].b_k"; zon1_roo_radTem_dummyGlaS351 "zon1.roo.radTem.dummyGlaSys.gas[1].a_mu"; zon1_roo_radTem_dummyGlaS352 "zon1.roo.radTem.dummyGlaSys.gas[1].b_mu"; zon1_roo_radTem_dummyGlaS353 "zon1.roo.radTem.dummyGlaSys.gas[1].a_c"; zon1_roo_radTem_dummyGlaS354 "zon1.roo.radTem.dummyGlaSys.gas[1].b_c"; zon1_roo_radTem_dummyGlaS355 "zon1.roo.radTem.dummyGlaSys.gas[1].MM"; zon1_roo_radTem_dummyGlaS356 "zon1.roo.radTem.dummyGlaSys.gas[1].P0"; zon1_roo_radTem_dummyGlaS357 "zon1.roo.radTem.dummyGlaSys.shade.tauSol_a"; zon1_roo_radTem_dummyGlaS358 "zon1.roo.radTem.dummyGlaSys.shade.tauSol_b"; zon1_roo_radTem_dummyGlaS359 "zon1.roo.radTem.dummyGlaSys.shade.rhoSol_a"; zon1_roo_radTem_dummyGlaS360 "zon1.roo.radTem.dummyGlaSys.shade.rhoSol_b"; zon1_roo_radTem_dummyGlaS361 "zon1.roo.radTem.dummyGlaSys.shade.absIR_a"; zon1_roo_radTem_dummyGlaS362 "zon1.roo.radTem.dummyGlaSys.shade.absIR_b"; zon1_roo_radTem_dummyGlaS363 "zon1.roo.radTem.dummyGlaSys.shade.tauIR_a"; zon1_roo_radTem_dummyGlaS364 "zon1.roo.radTem.dummyGlaSys.shade.tauIR_b"; zon1_roo_radTem_dummyGlaS365 "zon1.roo.radTem.dummyGlaSys.UFra"; zon1_roo_radTem_dummyGlaS366 "zon1.roo.radTem.dummyGlaSys.absIRFra"; zon1_roo_radTem_dummyGlaS367 "zon1.roo.radTem.dummyGlaSys.absSolFra"; zon1_roo_add_k1 "zon1.roo.add.k1"; zon1_roo_add_k2 "zon1.roo.add.k2"; zon1_roo_sumJFroWin_1__k "zon1.roo.sumJFroWin[1].k"; zon1_roo_p_start "zon1.roo.p_start"; zon1_roo_T_start "zon1.roo.T_start"; zon1_roo_X_start "zon1.roo.X_start"; zon1_qConGai_flow_k "zon1.qConGai_flow.k"; zon1_qRadGai_flow_k "zon1.qRadGai_flow.k"; zon1_qLatGai_flow_k "zon1.qLatGai_flow.k"; zon1_TSoi_1__T "zon1.TSoi[1].T"; zon1_sinInf_m_flow "zon1.sinInf.m_flow"; zon1_sinInf_x_pTphi_p "zon1.sinInf.x_pTphi.p"; zon1_InfiltrationRate_k "zon1.InfiltrationRate.k"; zon1_souInf_m_flow "zon1.souInf.m_flow"; zon1_souInf_x_pTphi_p "zon1.souInf.x_pTphi.p"; zon1_intLoad_table "zon1.intLoad.table"; zon1_intLoad_verboseRead "zon1.intLoad.verboseRead"; zon1_intLoad_columns "zon1.intLoad.columns"; zon1_intLoad_offset "zon1.intLoad.offset"; zon1_intLoad_startTime "zon1.intLoad.startTime"; zon1_intLoad_timeEvents "zon1.intLoad.timeEvents"; weaDat_pAtm "weaDat.pAtm"; weaDat_TDryBul "weaDat.TDryBul"; weaDat_TDewPoi "weaDat.TDewPoi"; weaDat_TBlaSky "weaDat.TBlaSky"; weaDat_relHum "weaDat.relHum"; weaDat_winSpe "weaDat.winSpe"; weaDat_winDir "weaDat.winDir"; weaDat_HInfHor "weaDat.HInfHor"; weaDat_ceiHei "weaDat.ceiHei"; weaDat_totSkyCov "weaDat.totSkyCov"; weaDat_opaSkyCov "weaDat.opaSkyCov"; weaDat_datRea_verboseRead "weaDat.datRea.verboseRead"; weaDat_cheTemDryBul_TMin "weaDat.cheTemDryBul.TMin"; weaDat_cheTemDryBul_TMax "weaDat.cheTemDryBul.TMax"; weaDat_cheTemDewPoi_TMin "weaDat.cheTemDewPoi.TMin"; weaDat_cheTemDewPoi_TMax "weaDat.cheTemDewPoi.TMax"; weaDat_add30Min_k1 "weaDat.add30Min.k1"; weaDat_add30Min_k2 "weaDat.add30Min.k2"; weaDat_datRea30Min_verbos407 "weaDat.datRea30Min.verboseRead"; weaDat_cheTemBlaSky_TMin "weaDat.cheTemBlaSky.TMin"; weaDat_cheTemBlaSky_TMax "weaDat.cheTemBlaSky.TMax"; rooSin_p "rooSin.p"; rooSin_T "rooSin.T"; rooSin_X "rooSin.X"; zon2_S_ "zon2.S_"; zon2_E_ "zon2.E_"; zon2_W_ "zon2.W_"; zon2_N_ "zon2.N_"; zon2_matExtWal_absIR_a "zon2.matExtWal.absIR_a"; zon2_matExtWal_absIR_b "zon2.matExtWal.absIR_b"; zon2_matExtWal_absSol_a "zon2.matExtWal.absSol_a"; zon2_matExtWal_absSol_b "zon2.matExtWal.absSol_b"; zon2_matExtWal_roughness_421 "zon2.matExtWal.roughness_a"; zon2_matFlo_absIR_a "zon2.matFlo.absIR_a"; zon2_matFlo_absIR_b "zon2.matFlo.absIR_b"; zon2_matFlo_absSol_a "zon2.matFlo.absSol_a"; zon2_matFlo_absSol_b "zon2.matFlo.absSol_b"; zon2_matFlo_roughness_a "zon2.matFlo.roughness_a"; zon2_roof_absIR_a "zon2.roof.absIR_a"; zon2_roof_absIR_b "zon2.roof.absIR_b"; zon2_roof_absSol_a "zon2.roof.absSol_a"; zon2_roof_absSol_b "zon2.roof.absSol_b"; zon2_roof_roughness_a "zon2.roof.roughness_a"; zon2_window600_glass_1__x "zon2.window600.glass[1].x"; zon2_window600_glass_1__k "zon2.window600.glass[1].k"; zon2_window600_glass_1__t434 "zon2.window600.glass[1].tauSol"; zon2_window600_glass_1__r435 "zon2.window600.glass[1].rhoSol_a"; zon2_window600_glass_1__r436 "zon2.window600.glass[1].rhoSol_b"; zon2_window600_glass_1__t437 "zon2.window600.glass[1].tauIR"; zon2_window600_glass_1__a438 "zon2.window600.glass[1].absIR_a"; zon2_window600_glass_1__a439 "zon2.window600.glass[1].absIR_b"; zon2_window600_glass_2__x "zon2.window600.glass[2].x"; zon2_window600_glass_2__k "zon2.window600.glass[2].k"; zon2_window600_glass_2__t442 "zon2.window600.glass[2].tauSol"; zon2_window600_glass_2__r443 "zon2.window600.glass[2].rhoSol_a"; zon2_window600_glass_2__r444 "zon2.window600.glass[2].rhoSol_b"; zon2_window600_glass_2__t445 "zon2.window600.glass[2].tauIR"; zon2_window600_glass_2__a446 "zon2.window600.glass[2].absIR_a"; zon2_window600_glass_2__a447 "zon2.window600.glass[2].absIR_b"; zon2_window600_gas_1__x "zon2.window600.gas[1].x"; zon2_window600_gas_1__a_k "zon2.window600.gas[1].a_k"; zon2_window600_gas_1__b_k "zon2.window600.gas[1].b_k"; zon2_window600_gas_1__a_m451 "zon2.window600.gas[1].a_mu"; zon2_window600_gas_1__b_m452 "zon2.window600.gas[1].b_mu"; zon2_window600_gas_1__a_c "zon2.window600.gas[1].a_c"; zon2_window600_gas_1__b_c "zon2.window600.gas[1].b_c"; zon2_window600_gas_1__MM "zon2.window600.gas[1].MM"; zon2_window600_gas_1__P0 "zon2.window600.gas[1].P0"; zon2_window600_shade_tauS457 "zon2.window600.shade.tauSol_a"; zon2_window600_shade_tauS458 "zon2.window600.shade.tauSol_b"; zon2_window600_shade_rhoS459 "zon2.window600.shade.rhoSol_a"; zon2_window600_shade_rhoS460 "zon2.window600.shade.rhoSol_b"; zon2_window600_shade_absI461 "zon2.window600.shade.absIR_a"; zon2_window600_shade_absI462 "zon2.window600.shade.absIR_b"; zon2_window600_shade_tauI463 "zon2.window600.shade.tauIR_a"; zon2_window600_shade_tauI464 "zon2.window600.shade.tauIR_b"; zon2_window600_UFra "zon2.window600.UFra"; zon2_window600_absIRFra "zon2.window600.absIRFra"; zon2_window600_absSolFra "zon2.window600.absSolFra"; zon2_soi_A "zon2.soi.A"; zon2_soi_T_a_start "zon2.soi.T_a_start"; zon2_soi_T_b_start "zon2.soi.T_b_start"; zon2_roo_datConExt_1__bou471 "zon2.roo.datConExt[1].boundaryCondition"; zon2_roo_datConExt_1__A "zon2.roo.datConExt[1].A"; zon2_roo_datConExt_2__bou473 "zon2.roo.datConExt[2].boundaryCondition"; zon2_roo_datConExt_2__A "zon2.roo.datConExt[2].A"; zon2_roo_datConExt_3__bou475 "zon2.roo.datConExt[3].boundaryCondition"; zon2_roo_datConExt_3__A "zon2.roo.datConExt[3].A"; zon2_roo_datConExt_4__bou477 "zon2.roo.datConExt[4].boundaryCondition"; zon2_roo_datConExt_4__A "zon2.roo.datConExt[4].A"; zon2_roo_datConExtWin_1__479 "zon2.roo.datConExtWin[1].boundaryCondition"; zon2_roo_datConExtWin_1__480 "zon2.roo.datConExtWin[1].A"; zon2_roo_datConExtWin_1__481 "zon2.roo.datConExtWin[1].hWin"; zon2_roo_datConExtWin_1__482 "zon2.roo.datConExtWin[1].wWin"; zon2_roo_datConExtWin_1__483 "zon2.roo.datConExtWin[1].fFra"; zon2_roo_datConExtWin_1__484 "zon2.roo.datConExtWin[1].ove.wL"; zon2_roo_datConExtWin_1__485 "zon2.roo.datConExtWin[1].ove.wR"; zon2_roo_datConExtWin_1__486 "zon2.roo.datConExtWin[1].ove.gap"; zon2_roo_datConExtWin_1__487 "zon2.roo.datConExtWin[1].sidFin.h"; zon2_roo_datConExtWin_1__488 "zon2.roo.datConExtWin[1].sidFin.gap"; zon2_roo_datConPar_1__azi "zon2.roo.datConPar[1].azi"; zon2_roo_datConPar_1__bou490 "zon2.roo.datConPar[1].boundaryCondition"; zon2_roo_datConPar_1__A "zon2.roo.datConPar[1].A"; zon2_roo_datConBou_1__azi "zon2.roo.datConBou[1].azi"; zon2_roo_datConBou_1__bou493 "zon2.roo.datConBou[1].boundaryCondition"; zon2_roo_datConBou_1__A "zon2.roo.datConBou[1].A"; zon2_roo_surBou_1__A "zon2.roo.surBou[1].A"; zon2_roo_surBou_1__absIR "zon2.roo.surBou[1].absIR"; zon2_roo_surBou_1__absSol "zon2.roo.surBou[1].absSol"; zon2_roo_surBou_1__bounda498 "zon2.roo.surBou[1].boundaryCondition"; zon2_roo_dummyCon_absIR_a "zon2.roo.dummyCon.absIR_a"; zon2_roo_dummyCon_absIR_b "zon2.roo.dummyCon.absIR_b"; zon2_roo_dummyCon_absSol_501 "zon2.roo.dummyCon.absSol_a"; zon2_roo_dummyCon_absSol_502 "zon2.roo.dummyCon.absSol_b"; zon2_roo_dummyCon_roughne503 "zon2.roo.dummyCon.roughness_a"; zon2_roo_dummyGlaSys_glas504 "zon2.roo.dummyGlaSys.glass[1].x"; zon2_roo_dummyGlaSys_glas505 "zon2.roo.dummyGlaSys.glass[1].k"; zon2_roo_dummyGlaSys_glas506 "zon2.roo.dummyGlaSys.glass[1].tauSol"; zon2_roo_dummyGlaSys_glas507 "zon2.roo.dummyGlaSys.glass[1].rhoSol_a"; zon2_roo_dummyGlaSys_glas508 "zon2.roo.dummyGlaSys.glass[1].rhoSol_b"; zon2_roo_dummyGlaSys_glas509 "zon2.roo.dummyGlaSys.glass[1].tauIR"; zon2_roo_dummyGlaSys_glas510 "zon2.roo.dummyGlaSys.glass[1].absIR_a"; zon2_roo_dummyGlaSys_glas511 "zon2.roo.dummyGlaSys.glass[1].absIR_b"; zon2_roo_dummyGlaSys_gas_512 "zon2.roo.dummyGlaSys.gas[1].x"; zon2_roo_dummyGlaSys_gas_513 "zon2.roo.dummyGlaSys.gas[1].a_k"; zon2_roo_dummyGlaSys_gas_514 "zon2.roo.dummyGlaSys.gas[1].b_k"; zon2_roo_dummyGlaSys_gas_515 "zon2.roo.dummyGlaSys.gas[1].a_mu"; zon2_roo_dummyGlaSys_gas_516 "zon2.roo.dummyGlaSys.gas[1].b_mu"; zon2_roo_dummyGlaSys_gas_517 "zon2.roo.dummyGlaSys.gas[1].a_c"; zon2_roo_dummyGlaSys_gas_518 "zon2.roo.dummyGlaSys.gas[1].b_c"; zon2_roo_dummyGlaSys_gas_519 "zon2.roo.dummyGlaSys.gas[1].MM"; zon2_roo_dummyGlaSys_gas_520 "zon2.roo.dummyGlaSys.gas[1].P0"; zon2_roo_dummyGlaSys_shad521 "zon2.roo.dummyGlaSys.shade.tauSol_a"; zon2_roo_dummyGlaSys_shad522 "zon2.roo.dummyGlaSys.shade.tauSol_b"; zon2_roo_dummyGlaSys_shad523 "zon2.roo.dummyGlaSys.shade.rhoSol_a"; zon2_roo_dummyGlaSys_shad524 "zon2.roo.dummyGlaSys.shade.rhoSol_b"; zon2_roo_dummyGlaSys_shad525 "zon2.roo.dummyGlaSys.shade.absIR_a"; zon2_roo_dummyGlaSys_shad526 "zon2.roo.dummyGlaSys.shade.absIR_b"; zon2_roo_dummyGlaSys_shad527 "zon2.roo.dummyGlaSys.shade.tauIR_a"; zon2_roo_dummyGlaSys_shad528 "zon2.roo.dummyGlaSys.shade.tauIR_b"; zon2_roo_dummyGlaSys_UFra "zon2.roo.dummyGlaSys.UFra"; zon2_roo_dummyGlaSys_absI530 "zon2.roo.dummyGlaSys.absIRFra"; zon2_roo_dummyGlaSys_absS531 "zon2.roo.dummyGlaSys.absSolFra"; zon2_roo_AFlo "zon2.roo.AFlo"; zon2_roo_hRoo "zon2.roo.hRoo"; zon2_roo_conExtWin_1__gla534 "zon2.roo.conExtWin[1].glaSys.haveControllableWindow"; zon2_roo_conExtWin_1__win535 "zon2.roo.conExtWin[1].win.matGla.k"; zon2_roo_conExtWin_1__win536 "zon2.roo.conExtWin[1].win.matGla.nStaRef"; zon2_roo_conExtWin_1__win537 "zon2.roo.conExtWin[1].win.matGla.piRef"; zon2_roo_conExtWin_1__win538 "zon2.roo.conExtWin[1].win.matGla.nStaReal"; zon2_roo_hIntFixed "zon2.roo.hIntFixed"; zon2_roo_hExtFixed "zon2.roo.hExtFixed"; zon2_roo_bouConExt_HDifTi541 "zon2.roo.bouConExt.HDifTil[1].rho"; zon2_roo_bouConExt_HDifTi542 "zon2.roo.bouConExt.HDifTil[1].add.k1"; zon2_roo_bouConExt_HDifTi543 "zon2.roo.bouConExt.HDifTil[1].add.k2"; zon2_roo_bouConExt_HDifTi544 "zon2.roo.bouConExt.HDifTil[2].rho"; zon2_roo_bouConExt_HDifTi545 "zon2.roo.bouConExt.HDifTil[2].add.k1"; zon2_roo_bouConExt_HDifTi546 "zon2.roo.bouConExt.HDifTil[2].add.k2"; zon2_roo_bouConExt_HDifTi547 "zon2.roo.bouConExt.HDifTil[3].rho"; zon2_roo_bouConExt_HDifTi548 "zon2.roo.bouConExt.HDifTil[3].add.k1"; zon2_roo_bouConExt_HDifTi549 "zon2.roo.bouConExt.HDifTil[3].add.k2"; zon2_roo_bouConExt_HDifTi550 "zon2.roo.bouConExt.HDifTil[4].rho"; zon2_roo_bouConExt_HDifTi551 "zon2.roo.bouConExt.HDifTil[4].add.k1"; zon2_roo_bouConExt_HDifTi552 "zon2.roo.bouConExt.HDifTil[4].add.k2"; zon2_roo_bouConExtWin_con553 "zon2.roo.bouConExtWin.conPar[1].ove.dep"; zon2_roo_bouConExtWin_con554 "zon2.roo.bouConExtWin.conPar[1].sidFin.dep"; zon2_roo_bouConExtWin_HDi555 "zon2.roo.bouConExtWin.HDifTil[1].rho"; zon2_roo_bouConExtWin_HDi556 "zon2.roo.bouConExtWin.HDifTil[1].add.k1"; zon2_roo_bouConExtWin_HDi557 "zon2.roo.bouConExtWin.HDifTil[1].add.k2"; zon2_roo_bouConExtWin_con558 "zon2.roo.bouConExtWin.conExtWin[1].radOut.T0"; zon2_roo_air_datConExtWin559 "zon2.roo.air.datConExtWin[1].ove.dep"; zon2_roo_air_datConExtWin560 "zon2.roo.air.datConExtWin[1].sidFin.dep"; zon2_roo_air_dummyCon_abs561 "zon2.roo.air.dummyCon.absIR_a"; zon2_roo_air_dummyCon_abs562 "zon2.roo.air.dummyCon.absIR_b"; zon2_roo_air_dummyCon_abs563 "zon2.roo.air.dummyCon.absSol_a"; zon2_roo_air_dummyCon_abs564 "zon2.roo.air.dummyCon.absSol_b"; zon2_roo_air_dummyCon_rou565 "zon2.roo.air.dummyCon.roughness_a"; zon2_roo_air_dummyGlaSys_566 "zon2.roo.air.dummyGlaSys.glass[1].x"; zon2_roo_air_dummyGlaSys_567 "zon2.roo.air.dummyGlaSys.glass[1].k"; zon2_roo_air_dummyGlaSys_568 "zon2.roo.air.dummyGlaSys.glass[1].tauSol"; zon2_roo_air_dummyGlaSys_569 "zon2.roo.air.dummyGlaSys.glass[1].rhoSol_a"; zon2_roo_air_dummyGlaSys_570 "zon2.roo.air.dummyGlaSys.glass[1].rhoSol_b"; zon2_roo_air_dummyGlaSys_571 "zon2.roo.air.dummyGlaSys.glass[1].tauIR"; zon2_roo_air_dummyGlaSys_572 "zon2.roo.air.dummyGlaSys.glass[1].absIR_a"; zon2_roo_air_dummyGlaSys_573 "zon2.roo.air.dummyGlaSys.glass[1].absIR_b"; zon2_roo_air_dummyGlaSys_574 "zon2.roo.air.dummyGlaSys.gas[1].x"; zon2_roo_air_dummyGlaSys_575 "zon2.roo.air.dummyGlaSys.gas[1].a_k"; zon2_roo_air_dummyGlaSys_576 "zon2.roo.air.dummyGlaSys.gas[1].b_k"; zon2_roo_air_dummyGlaSys_577 "zon2.roo.air.dummyGlaSys.gas[1].a_mu"; zon2_roo_air_dummyGlaSys_578 "zon2.roo.air.dummyGlaSys.gas[1].b_mu"; zon2_roo_air_dummyGlaSys_579 "zon2.roo.air.dummyGlaSys.gas[1].a_c"; zon2_roo_air_dummyGlaSys_580 "zon2.roo.air.dummyGlaSys.gas[1].b_c"; zon2_roo_air_dummyGlaSys_581 "zon2.roo.air.dummyGlaSys.gas[1].MM"; zon2_roo_air_dummyGlaSys_582 "zon2.roo.air.dummyGlaSys.gas[1].P0"; zon2_roo_air_dummyGlaSys_583 "zon2.roo.air.dummyGlaSys.shade.tauSol_a"; zon2_roo_air_dummyGlaSys_584 "zon2.roo.air.dummyGlaSys.shade.tauSol_b"; zon2_roo_air_dummyGlaSys_585 "zon2.roo.air.dummyGlaSys.shade.rhoSol_a"; zon2_roo_air_dummyGlaSys_586 "zon2.roo.air.dummyGlaSys.shade.rhoSol_b"; zon2_roo_air_dummyGlaSys_587 "zon2.roo.air.dummyGlaSys.shade.absIR_a"; zon2_roo_air_dummyGlaSys_588 "zon2.roo.air.dummyGlaSys.shade.absIR_b"; zon2_roo_air_dummyGlaSys_589 "zon2.roo.air.dummyGlaSys.shade.tauIR_a"; zon2_roo_air_dummyGlaSys_590 "zon2.roo.air.dummyGlaSys.shade.tauIR_b"; zon2_roo_air_dummyGlaSys_591 "zon2.roo.air.dummyGlaSys.UFra"; zon2_roo_air_dummyGlaSys_592 "zon2.roo.air.dummyGlaSys.absIRFra"; zon2_roo_air_dummyGlaSys_593 "zon2.roo.air.dummyGlaSys.absSolFra"; zon2_roo_solRadExc_datCon594 "zon2.roo.solRadExc.datConExtWin[1].ove.dep"; zon2_roo_solRadExc_datCon595 "zon2.roo.solRadExc.datConExtWin[1].sidFin.dep"; zon2_roo_solRadExc_dummyC596 "zon2.roo.solRadExc.dummyCon.absIR_a"; zon2_roo_solRadExc_dummyC597 "zon2.roo.solRadExc.dummyCon.absIR_b"; zon2_roo_solRadExc_dummyC598 "zon2.roo.solRadExc.dummyCon.absSol_a"; zon2_roo_solRadExc_dummyC599 "zon2.roo.solRadExc.dummyCon.absSol_b"; zon2_roo_solRadExc_dummyC600 "zon2.roo.solRadExc.dummyCon.roughness_a"; zon2_roo_solRadExc_dummyG601 "zon2.roo.solRadExc.dummyGlaSys.glass[1].x"; zon2_roo_solRadExc_dummyG602 "zon2.roo.solRadExc.dummyGlaSys.glass[1].k"; zon2_roo_solRadExc_dummyG603 "zon2.roo.solRadExc.dummyGlaSys.glass[1].tauSol"; zon2_roo_solRadExc_dummyG604 "zon2.roo.solRadExc.dummyGlaSys.glass[1].rhoSol_a"; zon2_roo_solRadExc_dummyG605 "zon2.roo.solRadExc.dummyGlaSys.glass[1].rhoSol_b"; zon2_roo_solRadExc_dummyG606 "zon2.roo.solRadExc.dummyGlaSys.glass[1].tauIR"; zon2_roo_solRadExc_dummyG607 "zon2.roo.solRadExc.dummyGlaSys.glass[1].absIR_a"; zon2_roo_solRadExc_dummyG608 "zon2.roo.solRadExc.dummyGlaSys.glass[1].absIR_b"; zon2_roo_solRadExc_dummyG609 "zon2.roo.solRadExc.dummyGlaSys.gas[1].x"; zon2_roo_solRadExc_dummyG610 "zon2.roo.solRadExc.dummyGlaSys.gas[1].a_k"; zon2_roo_solRadExc_dummyG611 "zon2.roo.solRadExc.dummyGlaSys.gas[1].b_k"; zon2_roo_solRadExc_dummyG612 "zon2.roo.solRadExc.dummyGlaSys.gas[1].a_mu"; zon2_roo_solRadExc_dummyG613 "zon2.roo.solRadExc.dummyGlaSys.gas[1].b_mu"; zon2_roo_solRadExc_dummyG614 "zon2.roo.solRadExc.dummyGlaSys.gas[1].a_c"; zon2_roo_solRadExc_dummyG615 "zon2.roo.solRadExc.dummyGlaSys.gas[1].b_c"; zon2_roo_solRadExc_dummyG616 "zon2.roo.solRadExc.dummyGlaSys.gas[1].MM"; zon2_roo_solRadExc_dummyG617 "zon2.roo.solRadExc.dummyGlaSys.gas[1].P0"; zon2_roo_solRadExc_dummyG618 "zon2.roo.solRadExc.dummyGlaSys.shade.tauSol_a"; zon2_roo_solRadExc_dummyG619 "zon2.roo.solRadExc.dummyGlaSys.shade.tauSol_b"; zon2_roo_solRadExc_dummyG620 "zon2.roo.solRadExc.dummyGlaSys.shade.rhoSol_a"; zon2_roo_solRadExc_dummyG621 "zon2.roo.solRadExc.dummyGlaSys.shade.rhoSol_b"; zon2_roo_solRadExc_dummyG622 "zon2.roo.solRadExc.dummyGlaSys.shade.absIR_a"; zon2_roo_solRadExc_dummyG623 "zon2.roo.solRadExc.dummyGlaSys.shade.absIR_b"; zon2_roo_solRadExc_dummyG624 "zon2.roo.solRadExc.dummyGlaSys.shade.tauIR_a"; zon2_roo_solRadExc_dummyG625 "zon2.roo.solRadExc.dummyGlaSys.shade.tauIR_b"; zon2_roo_solRadExc_dummyG626 "zon2.roo.solRadExc.dummyGlaSys.UFra"; zon2_roo_solRadExc_dummyG627 "zon2.roo.solRadExc.dummyGlaSys.absIRFra"; zon2_roo_solRadExc_dummyG628 "zon2.roo.solRadExc.dummyGlaSys.absSolFra"; zon2_roo_irRadGai_datConE629 "zon2.roo.irRadGai.datConExtWin[1].ove.dep"; zon2_roo_irRadGai_datConE630 "zon2.roo.irRadGai.datConExtWin[1].sidFin.dep"; zon2_roo_irRadGai_dummyCo631 "zon2.roo.irRadGai.dummyCon.absIR_a"; zon2_roo_irRadGai_dummyCo632 "zon2.roo.irRadGai.dummyCon.absIR_b"; zon2_roo_irRadGai_dummyCo633 "zon2.roo.irRadGai.dummyCon.absSol_a"; zon2_roo_irRadGai_dummyCo634 "zon2.roo.irRadGai.dummyCon.absSol_b"; zon2_roo_irRadGai_dummyCo635 "zon2.roo.irRadGai.dummyCon.roughness_a"; zon2_roo_irRadGai_dummyGl636 "zon2.roo.irRadGai.dummyGlaSys.glass[1].x"; zon2_roo_irRadGai_dummyGl637 "zon2.roo.irRadGai.dummyGlaSys.glass[1].k"; zon2_roo_irRadGai_dummyGl638 "zon2.roo.irRadGai.dummyGlaSys.glass[1].tauSol"; zon2_roo_irRadGai_dummyGl639 "zon2.roo.irRadGai.dummyGlaSys.glass[1].rhoSol_a"; zon2_roo_irRadGai_dummyGl640 "zon2.roo.irRadGai.dummyGlaSys.glass[1].rhoSol_b"; zon2_roo_irRadGai_dummyGl641 "zon2.roo.irRadGai.dummyGlaSys.glass[1].tauIR"; zon2_roo_irRadGai_dummyGl642 "zon2.roo.irRadGai.dummyGlaSys.glass[1].absIR_a"; zon2_roo_irRadGai_dummyGl643 "zon2.roo.irRadGai.dummyGlaSys.glass[1].absIR_b"; zon2_roo_irRadGai_dummyGl644 "zon2.roo.irRadGai.dummyGlaSys.gas[1].x"; zon2_roo_irRadGai_dummyGl645 "zon2.roo.irRadGai.dummyGlaSys.gas[1].a_k"; zon2_roo_irRadGai_dummyGl646 "zon2.roo.irRadGai.dummyGlaSys.gas[1].b_k"; zon2_roo_irRadGai_dummyGl647 "zon2.roo.irRadGai.dummyGlaSys.gas[1].a_mu"; zon2_roo_irRadGai_dummyGl648 "zon2.roo.irRadGai.dummyGlaSys.gas[1].b_mu"; zon2_roo_irRadGai_dummyGl649 "zon2.roo.irRadGai.dummyGlaSys.gas[1].a_c"; zon2_roo_irRadGai_dummyGl650 "zon2.roo.irRadGai.dummyGlaSys.gas[1].b_c"; zon2_roo_irRadGai_dummyGl651 "zon2.roo.irRadGai.dummyGlaSys.gas[1].MM"; zon2_roo_irRadGai_dummyGl652 "zon2.roo.irRadGai.dummyGlaSys.gas[1].P0"; zon2_roo_irRadGai_dummyGl653 "zon2.roo.irRadGai.dummyGlaSys.shade.tauSol_a"; zon2_roo_irRadGai_dummyGl654 "zon2.roo.irRadGai.dummyGlaSys.shade.tauSol_b"; zon2_roo_irRadGai_dummyGl655 "zon2.roo.irRadGai.dummyGlaSys.shade.rhoSol_a"; zon2_roo_irRadGai_dummyGl656 "zon2.roo.irRadGai.dummyGlaSys.shade.rhoSol_b"; zon2_roo_irRadGai_dummyGl657 "zon2.roo.irRadGai.dummyGlaSys.shade.absIR_a"; zon2_roo_irRadGai_dummyGl658 "zon2.roo.irRadGai.dummyGlaSys.shade.absIR_b"; zon2_roo_irRadGai_dummyGl659 "zon2.roo.irRadGai.dummyGlaSys.shade.tauIR_a"; zon2_roo_irRadGai_dummyGl660 "zon2.roo.irRadGai.dummyGlaSys.shade.tauIR_b"; zon2_roo_irRadGai_dummyGl661 "zon2.roo.irRadGai.dummyGlaSys.UFra"; zon2_roo_irRadGai_dummyGl662 "zon2.roo.irRadGai.dummyGlaSys.absIRFra"; zon2_roo_irRadGai_dummyGl663 "zon2.roo.irRadGai.dummyGlaSys.absSolFra"; zon2_roo_irRadExc_datConE664 "zon2.roo.irRadExc.datConExtWin[1].ove.dep"; zon2_roo_irRadExc_datConE665 "zon2.roo.irRadExc.datConExtWin[1].sidFin.dep"; zon2_roo_irRadExc_dummyCo666 "zon2.roo.irRadExc.dummyCon.absIR_a"; zon2_roo_irRadExc_dummyCo667 "zon2.roo.irRadExc.dummyCon.absIR_b"; zon2_roo_irRadExc_dummyCo668 "zon2.roo.irRadExc.dummyCon.absSol_a"; zon2_roo_irRadExc_dummyCo669 "zon2.roo.irRadExc.dummyCon.absSol_b"; zon2_roo_irRadExc_dummyCo670 "zon2.roo.irRadExc.dummyCon.roughness_a"; zon2_roo_irRadExc_dummyGl671 "zon2.roo.irRadExc.dummyGlaSys.glass[1].x"; zon2_roo_irRadExc_dummyGl672 "zon2.roo.irRadExc.dummyGlaSys.glass[1].k"; zon2_roo_irRadExc_dummyGl673 "zon2.roo.irRadExc.dummyGlaSys.glass[1].tauSol"; zon2_roo_irRadExc_dummyGl674 "zon2.roo.irRadExc.dummyGlaSys.glass[1].rhoSol_a"; zon2_roo_irRadExc_dummyGl675 "zon2.roo.irRadExc.dummyGlaSys.glass[1].rhoSol_b"; zon2_roo_irRadExc_dummyGl676 "zon2.roo.irRadExc.dummyGlaSys.glass[1].tauIR"; zon2_roo_irRadExc_dummyGl677 "zon2.roo.irRadExc.dummyGlaSys.glass[1].absIR_a"; zon2_roo_irRadExc_dummyGl678 "zon2.roo.irRadExc.dummyGlaSys.glass[1].absIR_b"; zon2_roo_irRadExc_dummyGl679 "zon2.roo.irRadExc.dummyGlaSys.gas[1].x"; zon2_roo_irRadExc_dummyGl680 "zon2.roo.irRadExc.dummyGlaSys.gas[1].a_k"; zon2_roo_irRadExc_dummyGl681 "zon2.roo.irRadExc.dummyGlaSys.gas[1].b_k"; zon2_roo_irRadExc_dummyGl682 "zon2.roo.irRadExc.dummyGlaSys.gas[1].a_mu"; zon2_roo_irRadExc_dummyGl683 "zon2.roo.irRadExc.dummyGlaSys.gas[1].b_mu"; zon2_roo_irRadExc_dummyGl684 "zon2.roo.irRadExc.dummyGlaSys.gas[1].a_c"; zon2_roo_irRadExc_dummyGl685 "zon2.roo.irRadExc.dummyGlaSys.gas[1].b_c"; zon2_roo_irRadExc_dummyGl686 "zon2.roo.irRadExc.dummyGlaSys.gas[1].MM"; zon2_roo_irRadExc_dummyGl687 "zon2.roo.irRadExc.dummyGlaSys.gas[1].P0"; zon2_roo_irRadExc_dummyGl688 "zon2.roo.irRadExc.dummyGlaSys.shade.tauSol_a"; zon2_roo_irRadExc_dummyGl689 "zon2.roo.irRadExc.dummyGlaSys.shade.tauSol_b"; zon2_roo_irRadExc_dummyGl690 "zon2.roo.irRadExc.dummyGlaSys.shade.rhoSol_a"; zon2_roo_irRadExc_dummyGl691 "zon2.roo.irRadExc.dummyGlaSys.shade.rhoSol_b"; zon2_roo_irRadExc_dummyGl692 "zon2.roo.irRadExc.dummyGlaSys.shade.absIR_a"; zon2_roo_irRadExc_dummyGl693 "zon2.roo.irRadExc.dummyGlaSys.shade.absIR_b"; zon2_roo_irRadExc_dummyGl694 "zon2.roo.irRadExc.dummyGlaSys.shade.tauIR_a"; zon2_roo_irRadExc_dummyGl695 "zon2.roo.irRadExc.dummyGlaSys.shade.tauIR_b"; zon2_roo_irRadExc_dummyGl696 "zon2.roo.irRadExc.dummyGlaSys.UFra"; zon2_roo_irRadExc_dummyGl697 "zon2.roo.irRadExc.dummyGlaSys.absIRFra"; zon2_roo_irRadExc_dummyGl698 "zon2.roo.irRadExc.dummyGlaSys.absSolFra"; zon2_roo_irRadExc_T0 "zon2.roo.irRadExc.T0"; zon2_roo_radTem_datConExt700 "zon2.roo.radTem.datConExtWin[1].ove.dep"; zon2_roo_radTem_datConExt701 "zon2.roo.radTem.datConExtWin[1].sidFin.dep"; zon2_roo_radTem_dummyCon_702 "zon2.roo.radTem.dummyCon.absIR_a"; zon2_roo_radTem_dummyCon_703 "zon2.roo.radTem.dummyCon.absIR_b"; zon2_roo_radTem_dummyCon_704 "zon2.roo.radTem.dummyCon.absSol_a"; zon2_roo_radTem_dummyCon_705 "zon2.roo.radTem.dummyCon.absSol_b"; zon2_roo_radTem_dummyCon_706 "zon2.roo.radTem.dummyCon.roughness_a"; zon2_roo_radTem_dummyGlaS707 "zon2.roo.radTem.dummyGlaSys.glass[1].x"; zon2_roo_radTem_dummyGlaS708 "zon2.roo.radTem.dummyGlaSys.glass[1].k"; zon2_roo_radTem_dummyGlaS709 "zon2.roo.radTem.dummyGlaSys.glass[1].tauSol"; zon2_roo_radTem_dummyGlaS710 "zon2.roo.radTem.dummyGlaSys.glass[1].rhoSol_a"; zon2_roo_radTem_dummyGlaS711 "zon2.roo.radTem.dummyGlaSys.glass[1].rhoSol_b"; zon2_roo_radTem_dummyGlaS712 "zon2.roo.radTem.dummyGlaSys.glass[1].tauIR"; zon2_roo_radTem_dummyGlaS713 "zon2.roo.radTem.dummyGlaSys.glass[1].absIR_a"; zon2_roo_radTem_dummyGlaS714 "zon2.roo.radTem.dummyGlaSys.glass[1].absIR_b"; zon2_roo_radTem_dummyGlaS715 "zon2.roo.radTem.dummyGlaSys.gas[1].x"; zon2_roo_radTem_dummyGlaS716 "zon2.roo.radTem.dummyGlaSys.gas[1].a_k"; zon2_roo_radTem_dummyGlaS717 "zon2.roo.radTem.dummyGlaSys.gas[1].b_k"; zon2_roo_radTem_dummyGlaS718 "zon2.roo.radTem.dummyGlaSys.gas[1].a_mu"; zon2_roo_radTem_dummyGlaS719 "zon2.roo.radTem.dummyGlaSys.gas[1].b_mu"; zon2_roo_radTem_dummyGlaS720 "zon2.roo.radTem.dummyGlaSys.gas[1].a_c"; zon2_roo_radTem_dummyGlaS721 "zon2.roo.radTem.dummyGlaSys.gas[1].b_c"; zon2_roo_radTem_dummyGlaS722 "zon2.roo.radTem.dummyGlaSys.gas[1].MM"; zon2_roo_radTem_dummyGlaS723 "zon2.roo.radTem.dummyGlaSys.gas[1].P0"; zon2_roo_radTem_dummyGlaS724 "zon2.roo.radTem.dummyGlaSys.shade.tauSol_a"; zon2_roo_radTem_dummyGlaS725 "zon2.roo.radTem.dummyGlaSys.shade.tauSol_b"; zon2_roo_radTem_dummyGlaS726 "zon2.roo.radTem.dummyGlaSys.shade.rhoSol_a"; zon2_roo_radTem_dummyGlaS727 "zon2.roo.radTem.dummyGlaSys.shade.rhoSol_b"; zon2_roo_radTem_dummyGlaS728 "zon2.roo.radTem.dummyGlaSys.shade.absIR_a"; zon2_roo_radTem_dummyGlaS729 "zon2.roo.radTem.dummyGlaSys.shade.absIR_b"; zon2_roo_radTem_dummyGlaS730 "zon2.roo.radTem.dummyGlaSys.shade.tauIR_a"; zon2_roo_radTem_dummyGlaS731 "zon2.roo.radTem.dummyGlaSys.shade.tauIR_b"; zon2_roo_radTem_dummyGlaS732 "zon2.roo.radTem.dummyGlaSys.UFra"; zon2_roo_radTem_dummyGlaS733 "zon2.roo.radTem.dummyGlaSys.absIRFra"; zon2_roo_radTem_dummyGlaS734 "zon2.roo.radTem.dummyGlaSys.absSolFra"; zon2_roo_add_k1 "zon2.roo.add.k1"; zon2_roo_add_k2 "zon2.roo.add.k2"; zon2_roo_sumJFroWin_1__k "zon2.roo.sumJFroWin[1].k"; zon2_roo_p_start "zon2.roo.p_start"; zon2_roo_T_start "zon2.roo.T_start"; zon2_roo_X_start "zon2.roo.X_start"; zon2_qConGai_flow_k "zon2.qConGai_flow.k"; zon2_qRadGai_flow_k "zon2.qRadGai_flow.k"; zon2_qLatGai_flow_k "zon2.qLatGai_flow.k"; zon2_TSoi_1__T "zon2.TSoi[1].T"; zon2_sinInf_m_flow "zon2.sinInf.m_flow"; zon2_sinInf_x_pTphi_p "zon2.sinInf.x_pTphi.p"; zon2_InfiltrationRate_k "zon2.InfiltrationRate.k"; zon2_souInf_m_flow "zon2.souInf.m_flow"; zon2_souInf_x_pTphi_p "zon2.souInf.x_pTphi.p"; zon2_intLoad_table "zon2.intLoad.table"; zon2_intLoad_verboseRead "zon2.intLoad.verboseRead"; zon2_intLoad_columns "zon2.intLoad.columns"; zon2_intLoad_offset "zon2.intLoad.offset"; zon2_intLoad_startTime "zon2.intLoad.startTime"; zon2_intLoad_timeEvents "zon2.intLoad.timeEvents"; vav2_vav_sta_default_p "vav2.vav.sta_default.p"; vav2_vav_sta_default_T "vav2.vav.sta_default.T"; vav2_vav_sta_default_X "vav2.vav.sta_default.X"; vav2_vav_riseTime "vav2.vav.riseTime"; vav2_vav_y_start "vav2.vav.y_start"; vav2_vav_filter_gain "vav2.vav.filter.gain"; vav2_vav_filter_A_ripple "vav2.vav.filter.A_ripple"; vav2_vav_filter_f_min "vav2.vav.filter.f_min"; vav2_vav_filter_normalize764 "vav2.vav.filter.normalized"; vav2_vav_filter_x_start "vav2.vav.filter.x_start"; vav2_vav_filter_u_nominal "vav2.vav.filter.u_nominal"; vav2_vav_use_deltaM "vav2.vav.use_deltaM"; vav2_vav_deltaM "vav2.vav.deltaM"; vav2_vav_roundDuct "vav2.vav.roundDuct"; vav2_vav_ReC "vav2.vav.ReC"; vav2_vav_a "vav2.vav.a"; vav2_vav_b "vav2.vav.b"; vav2_vav_yL "vav2.vav.yL"; vav2_vav_yU "vav2.vav.yU"; vav2_vav_k1 "vav2.vav.k1"; vav2_vav_l "vav2.vav.l"; vav2_vav_l2 "vav2.vav.l2"; vav2_vav_deltax "vav2.vav.deltax"; vav2_vav_y_min "vav2.vav.y_min"; vav2_terHea_bal1_preDro_s780 "vav2.terHea.bal1.preDro.sta_default.p"; vav2_terHea_bal1_preDro_s781 "vav2.terHea.bal1.preDro.sta_default.T"; vav2_terHea_bal1_preDro_s782 "vav2.terHea.bal1.preDro.sta_default.X"; vav2_terHea_bal2_preDro_s783 "vav2.terHea.bal2.preDro.sta_default.p"; vav2_terHea_bal2_preDro_s784 "vav2.terHea.bal2.preDro.sta_default.T"; vav2_terHea_delta "vav2.terHea.delta"; vav2_terHea_T_a1_nominal "vav2.terHea.T_a1_nominal"; vav2_terHea_T_a2_nominal "vav2.terHea.T_a2_nominal"; vav2_terHea_r_nominal "vav2.terHea.r_nominal"; vav2_terHea_hA_n_w "vav2.terHea.hA.n_w"; vav2_terHea_hA_n_a "vav2.terHea.hA.n_a"; vav2_terHea_hA_T0_w "vav2.terHea.hA.T0_w"; vav2_terHea_hA_T0_a "vav2.terHea.hA.T0_a"; vav2_sinTer_X "vav2.sinTer.X"; vav2_sinTer_p "vav2.sinTer.p"; vav2_sinTer_T "vav2.sinTer.T"; vav2_souTer_X "vav2.souTer.X"; vav2_souTer_m_flow "vav2.souTer.m_flow"; vav2_souTer_T "vav2.souTer.T"; coiSou_X "coiSou.X"; coiSou_T "coiSou.T"; byp_sta_default_p "byp.sta_default.p"; byp_sta_default_T "byp.sta_default.T"; byp_sta_default_X "byp.sta_default.X"; VSup2_T_start "VSup2.T_start"; VSup2_p_start "VSup2.p_start"; VSup2_X_start "VSup2.X_start"; VSup1_T_start "VSup1.T_start"; VSup1_p_start "VSup1.p_start"; VSup1_X_start "VSup1.X_start"; TDisVAV1_T_start "TDisVAV1.T_start"; TDisVAV1_TAmb "TDisVAV1.TAmb"; TDisVAV1_tauHeaTra "TDisVAV1.tauHeaTra"; TDisVAV2_T_start "TDisVAV2.T_start"; TDisVAV2_TAmb "TDisVAV2.TAmb"; TDisVAV2_tauHeaTra "TDisVAV2.tauHeaTra"; zon1_roo_conExtWin_1__win816 "zon1.roo.conExtWin[1].win.glaUns.glass[1].T0"; zon1_roo_conExtWin_1__win817 "zon1.roo.conExtWin[1].win.glaUns.glass[2].T0"; zon1_roo_conExtWin_1__win818 "zon1.roo.conExtWin[1].win.glaUns.gas[1].T0"; zon2_roo_conExtWin_1__win819 "zon2.roo.conExtWin[1].win.glaUns.glass[1].T0"; zon2_roo_conExtWin_1__win820 "zon2.roo.conExtWin[1].win.glaUns.glass[2].T0"; zon2_roo_conExtWin_1__win821 "zon2.roo.conExtWin[1].win.glaUns.gas[1].T0"
      mask Display: image(imread('Dymola.bmp'))
  compmodel : Subsystem
      settings: OpenFcn=compileModelica('ds_simple_twozone/behavior/DymolaBlock');
      mask Display: disp('Compile Modelica model');
  editmodel : Subsystem
      settings: OpenFcn=editModelica('ds_simple_twozone/behavior/DymolaBlock');
      mask Display: disp('Edit Modelica model');
  V2_flow : Outport
  V1_flow : Outport  Port=2
  TRooAir2 : Outport  Port=3
  TRooAir1 : Outport  Port=4
  TDis2 : Outport  Port=5
  TDis1 : Outport  Port=6
  weaBus_HDifHor : Outport  Port=7
  weaBus_HDirNor : Outport  Port=8
  weaBus_HGloHor : Outport  Port=9
  weaBus_HHorIR : Outport  Port=10
  weaBus_TBlaSky : Outport  Port=11
  weaBus_TDewPoi : Outport  Port=12
  weaBus_TDryBul : Outport  Port=13
  weaBus_ceiHei : Outport  Port=14
  weaBus_cloTim : Outport  Port=15
  weaBus_lat : Outport  Port=16
  weaBus_lon : Outport  Port=17
  weaBus_nOpa : Outport  Port=18
  weaBus_nTot : Outport  Port=19
  weaBus_pAtm : Outport  Port=20
  weaBus_relHum : Outport  Port=21
  weaBus_solAlt : Outport  Port=22
  weaBus_solDec : Outport  Port=23
  weaBus_solHouAng : Outport  Port=24
  weaBus_solTim : Outport  Port=25
  weaBus_solZen : Outport  Port=26
  weaBus_winDir : Outport  Port=27
  weaBus_winSpe : Outport  Port=28
  wires:
  Sfunc/1 -> Demux/1
  Demux/1 -> V2_flow/1
  Demux/2 -> V1_flow/1
  Demux/3 -> TRooAir2/1
  Demux/4 -> TRooAir1/1
  Demux/5 -> TDis2/1
  Demux/6 -> TDis1/1
  Demux/7 -> weaBus_HDifHor/1
  Demux/8 -> weaBus_HDirNor/1
  Demux/9 -> weaBus_HGloHor/1
  Demux/10 -> weaBus_HHorIR/1
  Demux/11 -> weaBus_TBlaSky/1
  Demux/12 -> weaBus_TDewPoi/1
  Demux/13 -> weaBus_TDryBul/1
  Demux/14 -> weaBus_ceiHei/1
  Demux/15 -> weaBus_cloTim/1
  Demux/16 -> weaBus_lat/1
  Demux/17 -> weaBus_lon/1
  Demux/18 -> weaBus_nOpa/1
  Demux/19 -> weaBus_nTot/1
  Demux/20 -> weaBus_pAtm/1
  Demux/21 -> weaBus_relHum/1
  Demux/22 -> weaBus_solAlt/1
  Demux/23 -> weaBus_solDec/1
  Demux/24 -> weaBus_solHouAng/1
  Demux/25 -> weaBus_solTim/1
  Demux/26 -> weaBus_solZen/1
  Demux/27 -> weaBus_winDir/1
  Demux/28 -> weaBus_winSpe/1
  Mux/1 -> Sfunc/1
  yVAV1/1 -> Mux/1
  yVAV2/1 -> Mux/2
